simulink library "outp"  (R2021b)
(part 7 of 7)

  VNMM_NetworkReq_flg/1 -> VNMM_NetworkReq_flg_Inproc/1  "VNMM_NetworkReq_flg"
  VNMM_NetworkReq_flg_Inproc/1 -> UnitConverter226/1
  UnitConverter226/1 -> VOUTP_NetworkReq_flg/1  "VOUTP_NetworkReq_flg"
  VPMM_PowerUpState_enum/1 -> VPMM_PowerUpState_enum_Inproc/1  "VPMM_PowerUpState_enum"
  VPMM_PowerUpState_enum_Inproc/1 -> UnitConverter227/1
  UnitConverter227/1 -> VOUTP_PowerUpState_enum/1  "VOUTP_PowerUpState_enum"
  VPMM_PowerDownState_enum/1 -> VPMM_PowerDownState_enum_Inproc/1  "VPMM_PowerDownState_enum"
  VPMM_PowerDownState_enum_Inproc/1 -> UnitConverter228/1
  UnitConverter228/1 -> VOUTP_PowerDownState_enum/1  "VOUTP_PowerDownState_enum"
  VPMM_PowerUpFault_enum/1 -> VPMM_PowerUpFault_enum_Inproc/1  "VPMM_PowerUpFault_enum"
  VPMM_PowerUpFault_enum_Inproc/1 -> UnitConverter229/1
  UnitConverter229/1 -> VOUTP_PowerUpFault_enum/1  "VOUTP_PowerUpFault_enum"
  VPMM_PowerDownFault_enum/1 -> VPMM_PowerDownFault_enum_Inproc/1  "VPMM_PowerDownFault_enum"
  VPMM_PowerDownFault_enum_Inproc/1 -> UnitConverter230/1
  UnitConverter230/1 -> VOUTP_PowerDownFault_enum/1  "VOUTP_PowerDownFault_enum"
  VPMM_ActiveDischargeReq_flg/1 -> VPMM_ActiveDischargeReq_flg_Inproc/1  "VPMM_ActiveDischargeReq_flg"
  VPMM_ActiveDischargeReq_flg_Inproc/1 -> UnitConverter231/1
  UnitConverter231/1 -> VOUTP_ActiveDischargeReq_flg/1  "VOUTP_ActiveDischargeReq_flg"
  VPMM_DCDCEnaReq_flg/1 -> VPMM_DCDCEnaReq_flg_Inproc/1  "VPMM_DCDCEnaReq_flg"
  VPMM_DCDCEnaReq_flg_Inproc/1 -> UnitConverter232/1
  UnitConverter232/1 -> VOUTP_DCDCEnaReq_flg/1  "VOUTP_DCDCEnaReq_flg"
  VPMM_DCDCVoltSetpoint_V/1 -> VPMM_DCDCVoltSetpoint_V_Inproc/1  "VPMM_DCDCVoltSetpoint_V"
  VPMM_DCDCVoltSetpoint_V_Inproc/1 -> UnitConverter233/1
  UnitConverter233/1 -> VOUTP_DCDCVoltSetpoint_V/1  "VOUTP_DCDCVoltSetpoint_V"
  VPMM_HVBatCnctReq_flg/1 -> VPMM_HVBatCnctReq_flg_Inproc/1  "VPMM_HVBatCnctReq_flg"
  VPMM_HVBatCnctReq_flg_Inproc/1 -> UnitConverter234/1
  UnitConverter234/1 -> VOUTP_HVBatCnctReq_flg/1  "VOUTP_HVBatCnctReq_flg"
  VPMM_HVSysReadyToCharge_enum/1 -> VPMM_HVSysReadyToCharge_enum_Inproc/1  "VPMM_HVSysReadyToCharge_enum"
  VPMM_HVSysReadyToCharge_enum_Inproc/1 -> UnitConverter235/1
  UnitConverter235/1 -> VOUTP_HVSysReadyToCharge_enum/1  "VOUTP_HVSysReadyToCharge_enum"
  VPMM_PowerSta_enum/1 -> VPMM_PowerSta_enum_Inproc/1  "VPMM_PowerSta_enum"
  VPMM_PowerSta_enum_Inproc/1 -> UnitConverter236/1
  UnitConverter236/1 -> VOUTP_PowerSta_enum/1  "VOUTP_PowerSta_enum"
  VPMM_LVPwrSta_flg/1 -> VPMM_LVPwrSta_flg_Inproc/1  "VPMM_LVPwrSta_flg"
  VPMM_LVPwrSta_flg_Inproc/1 -> UnitConverter237/1
  UnitConverter237/1 -> VOUTP_LVPwrSta_flg/1  "VOUTP_LVPwrSta_flg"
  VPMM_HVPwrSta_flg/1 -> VPMM_HVPwrSta_flg_Inproc/1  "VPMM_HVPwrSta_flg"
  VPMM_HVPwrSta_flg_Inproc/1 -> UnitConverter238/1
  UnitConverter238/1 -> VOUTP_HVPwrSta_flg/1  "VOUTP_HVPwrSta_flg"
  VPMM_SysPowerMode_enum/1 -> VPMM_SysPowerMode_enum_Inproc/1  "VPMM_SysPowerMode_enum"
  VPMM_SysPowerMode_enum_Inproc/1 -> UnitConverter239/1
  UnitConverter239/1 -> VOUTP_SysPowerMode_enum/1  "VOUTP_SysPowerMode_enum"
  VPMM_FrMCUEnaReq_flg/1 -> VPMM_FrMCUEnaReq_flg_Inproc/1  "VPMM_FrMCUEnaReq_flg"
  VPMM_FrMCUEnaReq_flg_Inproc/1 -> UnitConverter240/1
  UnitConverter240/1 -> VOUTP_FrMCUEnaReq_flg/1  "VOUTP_FrMCUEnaReq_flg"
  VPMM_RrMCUEnaReq_flg/1 -> VPMM_RrMCUEnaReq_flg_Inproc/1  "VPMM_RrMCUEnaReq_flg"
  VPMM_RrMCUEnaReq_flg_Inproc/1 -> UnitConverter241/1
  UnitConverter241/1 -> VOUTP_RrMCUEnaReq_flg/1  "VOUTP_RrMCUEnaReq_flg"
  VPMM_DrivetrainSelect_enum/1 -> VPMM_DrivetrainSelect_enum_Inproc/1  "VPMM_DrivetrainSelect_enum"
  VPMM_DrivetrainSelect_enum_Inproc/1 -> UnitConverter242/1
  UnitConverter242/1 -> VOUTP_DrivetrainSelect_enum/1  "VOUTP_DrivetrainSelect_enum"
  VPMM_DrSeatSta_enum/1 -> VPMM_DrSeatSta_enum_Inproc/1  "VPMM_DrSeatSta_enum"
  VPMM_DrSeatSta_enum_Inproc/1 -> UnitConverter243/1
  UnitConverter243/1 -> VOUTP_DrSeatSta_enum/1  "VOUTP_DrSeatSta_enum"
  VPMM_PwrStaSelect_enum/1 -> VPMM_PwrStaSelect_enum_Inproc/1  "VPMM_PwrStaSelect_enum"
  VPMM_PwrStaSelect_enum_Inproc/1 -> UnitConverter244/1
  UnitConverter244/1 -> VOUTP_PwrStaSelect_enum/1  "VOUTP_PwrStaSelect_enum"
  VPMM_PwrStaConstraint_enum/1 -> VPMM_PwrStaConstraint_enum_Inproc/1  "VPMM_PwrStaConstraint_enum"
  VPMM_PwrStaConstraint_enum_Inproc/1 -> UnitConverter245/1
  UnitConverter245/1 -> VOUTP_PwrStaConstraint_enum/1  "VOUTP_PwrStaConstraint_enum"
  VPMM_TCountSta_enum/1 -> VPMM_TCountSta_enum_Inproc/1  "VPMM_TCountSta_enum"
  VPMM_TCountSta_enum_Inproc/1 -> UnitConverter246/1
  UnitConverter246/1 -> VOUTP_TCountSta_enum/1  "VOUTP_TCountSta_enum"
  VPMM_PwrUpReq_enum/1 -> VPMM_PwrUpReq_enum_Inproc/1  "VPMM_PwrUpReq_enum"
  VPMM_PwrUpReq_enum_Inproc/1 -> UnitConverter247/1
  UnitConverter247/1 -> VOUTP_PwrUpReq_enum/1  "VOUTP_PwrUpReq_enum"
  VPMM_PwrDownReq_enum/1 -> VPMM_PwrDownReq_enum_Inproc/1  "VPMM_PwrDownReq_enum"
  VPMM_PwrDownReq_enum_Inproc/1 -> UnitConverter248/1
  UnitConverter248/1 -> VOUTP_PwrDownReq_enum/1  "VOUTP_PwrDownReq_enum"
  VPMM_LowSOCWarn_enum/1 -> VPMM_LowSOCWarn_enum_Inproc/1  "VPMM_LowSOCWarn_enum"
  VPMM_LowSOCWarn_enum_Inproc/1 -> UnitConverter249/1
  UnitConverter249/1 -> VOUTP_LowSOCWarn_enum/1  "VOUTP_LowSOCWarn_enum"
  VPMM_ReVehThdChkSta_enum/1 -> VPMM_ReVehThdChkSta_enum_Inproc/1  "VPMM_ReVehThdChkSta_enum"
  VPMM_ReVehThdChkSta_enum_Inproc/1 -> UnitConverter250/1
  UnitConverter250/1 -> VOUTP_ReVehThdChkSta_enum/1  "VOUTP_ReVehThdChkSta_enum"
  VPMM_LVSysErrPwrOutErr_flg/1 -> VPMM_LVSysErrPwrOutErr_flg_Inproc/1  "VPMM_LVSysErrPwrOutErr_flg"
  VPMM_LVSysErrPwrOutErr_flg_Inproc/1 -> UnitConverter251/1
  UnitConverter251/1 -> VOUTP_LVSysErrPwrOutErr_flg/1  "VOUTP_LVSysErrPwrOutErr_flg"
  VPMM_EvccAplusPwrUpReq_flg/1 -> VPMM_EvccAplusPwrUpReq_flg_Inproc/1  "VPMM_EvccAplusPwrUpReq_flg"
  VPMM_EvccAplusPwrUpReq_flg_Inproc/1 -> UnitConverter252/1
  UnitConverter252/1 -> VOUTP_EvccAplusPwrUpReq_flg/1  "VOUTP_EvccAplusPwrUpReq_flg"
  VPMM_PwrStaONTOPopReq_flg/1 -> VPMM_PwrStaONTOPopReq_flg_Inproc/1  "VPMM_PwrStaONTOPopReq_flg"
  VPMM_PwrStaONTOPopReq_flg_Inproc/1 -> UnitConverter253/1
  UnitConverter253/1 -> VOUTP_PwrStaONTOPopReq_flg/1  "VOUTP_PwrStaONTOPopReq_flg"
  VPMM_IVIPwrStaONTOPopT_s/1 -> VPMM_IVIPwrStaONTOPopT_s_Inproc/1  "VPMM_IVIPwrStaONTOPopT_s"
  VPMM_IVIPwrStaONTOPopT_s_Inproc/1 -> UnitConverter254/1
  UnitConverter254/1 -> VOUTP_IVIPwrStaONTOPopT_s/1  "VOUTP_IVIPwrStaONTOPopT_s"
  VPMM_LVChrgHoldTtimer_s/1 -> VPMM_LVChrgHoldTtimer_s_Inproc/1  "VPMM_LVChrgHoldTtimer_s"
  VPMM_LVChrgHoldTtimer_s_Inproc/1 -> UnitConverter255/1
  UnitConverter255/1 -> VOUTP_LVChrgHoldTtimer_s/1  "VOUTP_LVChrgHoldTtimer_s"
  VPMM_LVBattChrgTimeCnt_s/1 -> VPMM_LVBattChrgTimeCnt_s_Inproc/1  "VPMM_LVBattChrgTimeCnt_s"
  VPMM_LVBattChrgTimeCnt_s_Inproc/1 -> UnitConverter256/1
  UnitConverter256/1 -> VOUTP_LVBattChrgTimeCnt_s/1  "VOUTP_LVBattChrgTimeCnt_s"
  VPMM_SilentChkAllowSleep_flg/1 -> VPMM_SilentChkAllowSleep_flg_Inproc/1  "VPMM_SilentChkAllowSleep_flg"
  VPMM_SilentChkAllowSleep_flg_Inproc/1 -> UnitConverter257/1
  UnitConverter257/1 -> VOUTP_SilentChkAllowSleep_flg/1  "VOUTP_SilentChkAllowSleep_flg"
  VPMM_TimerAllowSleep_flg/1 -> VPMM_TimerAllowSleep_flg_Inproc/1  "VPMM_TimerAllowSleep_flg"
  VPMM_TimerAllowSleep_flg_Inproc/1 -> UnitConverter258/1
  UnitConverter258/1 -> VOUTP_TimerAllowSleep_flg/1  "VOUTP_TimerAllowSleep_flg"
  VPMM_FDADC12VDetAvg_mV/1 -> VPMM_FDADC12VDetAvg_mV_Inproc/1  "VPMM_FDADC12VDetAvg_mV"
  VPMM_FDADC12VDetAvg_mV_Inproc/1 -> UnitConverter259/1
  UnitConverter259/1 -> VOUTP_FDADC12VDetAvg_mV/1  "VOUTP_FDADC12VDetAvg_mV"
  VPMM_PMMAllowECUSleep_flg/1 -> VPMM_PMMAllowECUSleep_flg_Inproc/1  "VPMM_PMMAllowECUSleep_flg"
  VPMM_PMMAllowECUSleep_flg_Inproc/1 -> UnitConverter260/1
  UnitConverter260/1 -> VOUTP_PMMAllowECUSleep_flg/1  "VOUTP_PMMAllowECUSleep_flg"
  VPMM_LVSilentChrgSta_enum/1 -> VPMM_LVSilentChrgSta_enum_Inproc/1  "VPMM_LVSilentChrgSta_enum"
  VPMM_LVSilentChrgSta_enum_Inproc/1 -> UnitConverter261/1
  UnitConverter261/1 -> VOUTP_LVSilentChrgSta_enum/1  "VOUTP_LVSilentChrgSta_enum"
  VPMM_LVSilentChrgReq_flg/1 -> VPMM_LVSilentChrgReq_flg_Inproc/1  "VPMM_LVSilentChrgReq_flg"
  VPMM_LVSilentChrgReq_flg_Inproc/1 -> UnitConverter262/1
  UnitConverter262/1 -> VOUTP_LVSilentChrgReq_flg/1  "VOUTP_LVSilentChrgReq_flg"
  VPMM_LVSilentChrgLv_enum/1 -> VPMM_LVSilentChrgLv_enum_Inproc/1  "VPMM_LVSilentChrgLv_enum"
  VPMM_LVSilentChrgLv_enum_Inproc/1 -> UnitConverter263/1
  UnitConverter263/1 -> VOUTP_LVSilentChrgLv_enum/1  "VOUTP_LVSilentChrgLv_enum"
  VPMM_CtrlFrPwrStbA1P_flg/1 -> VPMM_CtrlFrPwrStbA1P_flg_Inproc/1  "VPMM_CtrlFrPwrStbA1P_flg"
  VPMM_CtrlFrPwrStbA1P_flg_Inproc/1 -> UnitConverter264/1
  UnitConverter264/1 -> VOUTP_CtrlFrPwrStbA1P_flg/1  "VOUTP_CtrlFrPwrStbA1P_flg"
  VPMM_CtrlFrRC1_flg/1 -> VPMM_CtrlFrRC1_flg_Inproc/1  "VPMM_CtrlFrRC1_flg"
  VPMM_CtrlFrRC1_flg_Inproc/1 -> UnitConverter265/1
  UnitConverter265/1 -> VOUTP_CtrlFrRC1_flg/1  "VOUTP_CtrlFrRC1_flg"
  VPMM_CtrlFrBMSCCUCIR_flg/1 -> VPMM_CtrlFrBMSCCUCIR_flg_Inproc/1  "VPMM_CtrlFrBMSCCUCIR_flg"
  VPMM_CtrlFrBMSCCUCIR_flg_Inproc/1 -> UnitConverter266/1
  UnitConverter266/1 -> VOUTP_CtrlFrBMSCCUCIR_flg/1  "VOUTP_CtrlFrBMSCCUCIR_flg"
  VPMM_CtrlFrEDUINVERTER_flg/1 -> VPMM_CtrlFrEDUINVERTER_flg_Inproc/1  "VPMM_CtrlFrEDUINVERTER_flg"
  VPMM_CtrlFrEDUINVERTER_flg_Inproc/1 -> UnitConverter267/1
  UnitConverter267/1 -> VOUTP_CtrlFrEDUINVERTER_flg/1  "VOUTP_CtrlFrEDUINVERTER_flg"
  VPMM_HWResetSta_enum/1 -> VPMM_HWResetSta_enum_Inproc/1  "VPMM_HWResetSta_enum"
  VPMM_HWResetSta_enum_Inproc/1 -> UnitConverter268/1
  UnitConverter268/1 -> VOUTP_HWResetSta_enum/1  "VOUTP_HWResetSta_enum"
  VPMM_CtrlDrPwrStbA2_flg/1 -> VPMM_CtrlDrPwrStbA2_flg_Inproc/1  "VPMM_CtrlDrPwrStbA2_flg"
  VPMM_CtrlDrPwrStbA2_flg_Inproc/1 -> UnitConverter269/1
  UnitConverter269/1 -> VOUTP_CtrlDrPwrStbA2_flg/1  "VOUTP_CtrlDrPwrStbA2_flg"
  VPMM_PwrStaTOSta_enum/1 -> VPMM_PwrStaTOSta_enum_Inproc/1  "VPMM_PwrStaTOSta_enum"
  VPMM_PwrStaTOSta_enum_Inproc/1 -> UnitConverter270/1
  UnitConverter270/1 -> VOUTP_PwrStaTOSta_enum/1  "VOUTP_PwrStaTOSta_enum"
  VPMM_DCDCRlyDem_enum/1 -> VPMM_DCDCRlyDem_enum_Inproc/1  "VPMM_DCDCRlyDem_enum"
  VPMM_DCDCRlyDem_enum_Inproc/1 -> UnitConverter271/1
  UnitConverter271/1 -> VOUTP_DCDCRlyDem_enum/1  "VOUTP_DCDCRlyDem_enum"
  VPMM_EACRlyDem_enum/1 -> VPMM_EACRlyDem_enum_Inproc/1  "VPMM_EACRlyDem_enum"
  VPMM_EACRlyDem_enum_Inproc/1 -> UnitConverter272/1
  UnitConverter272/1 -> VOUTP_EACRlyDem_enum/1  "VOUTP_EACRlyDem_enum"
  VPMM_EHPSRlyDem_enum/1 -> VPMM_EHPSRlyDem_enum_Inproc/1  "VPMM_EHPSRlyDem_enum"
  VPMM_EHPSRlyDem_enum_Inproc/1 -> UnitConverter273/1
  UnitConverter273/1 -> VOUTP_EHPSRlyDem_enum/1  "VOUTP_EHPSRlyDem_enum"
  VPMM_DCDCEnDem_enum/1 -> VPMM_DCDCEnDem_enum_Inproc/1  "VPMM_DCDCEnDem_enum"
  VPMM_DCDCEnDem_enum_Inproc/1 -> UnitConverter274/1
  UnitConverter274/1 -> VOUTP_DCDCEnDem_enum/1  "VOUTP_DCDCEnDem_enum"
  VSCP_Vehspeed_kph/1 -> VSCP_Vehspeed_kph_Inproc/1  "VSCP_Vehspeed_kph"
  VSCP_Vehspeed_kph_Inproc/1 -> UnitConverter275/1
  UnitConverter275/1 -> VOUTP_Vehspeed_kph/1  "VOUTP_Vehspeed_kph"
  VSCP_SCPBrkSwSta_flg/1 -> VSCP_SCPBrkSwSta_flg_Inproc/1  "VSCP_SCPBrkSwSta_flg"
  VSCP_SCPBrkSwSta_flg_Inproc/1 -> UnitConverter276/1
  UnitConverter276/1 -> VOUTP_SCPBrkSwSta_flg/1  "VOUTP_SCPBrkSwSta_flg"
  VSCP_AmberWnlmpSta_flg/1 -> VSCP_AmberWnlmpSta_flg_Inproc/1  "VSCP_AmberWnlmpSta_flg"
  VSCP_AmberWnlmpSta_flg_Inproc/1 -> UnitConverter277/1
  UnitConverter277/1 -> VOUTP_AmberWnlmpSta_flg/1  "VOUTP_AmberWnlmpSta_flg"
  VSCP_ABSWnlmpSta_flg/1 -> VSCP_ABSWnlmpSta_flg_Inproc/1  "VSCP_ABSWnlmpSta_flg"
  VSCP_ABSWnlmpSta_flg_Inproc/1 -> UnitConverter278/1
  UnitConverter278/1 -> VOUTP_ABSWnlmpSta_flg/1  "VOUTP_ABSWnlmpSta_flg"
  VSCP_HSAFailed_flg/1 -> VSCP_HSAFailed_flg_Inproc/1  "VSCP_HSAFailed_flg"
  VSCP_HSAFailed_flg_Inproc/1 -> UnitConverter279/1
  UnitConverter279/1 -> VOUTP_HSAFailed_flg/1  "VOUTP_HSAFailed_flg"
  VSCP_MeterIndVehSpeed_kph/1 -> VSCP_MeterIndVehSpeed_kph_Inproc/1  "VSCP_MeterIndVehSpeed_kph"
  VSCP_MeterIndVehSpeed_kph_Inproc/1 -> UnitConverter280/1
  UnitConverter280/1 -> VOUTP_MeterIndVehSpeed_kph/1  "VOUTP_MeterIndVehSpeed_kph"
  VSCP_ABSFailed_flg/1 -> VSCP_ABSFailed_flg_Inproc/1  "VSCP_ABSFailed_flg"
  VSCP_ABSFailed_flg_Inproc/1 -> UnitConverter281/1
  UnitConverter281/1 -> VOUTP_ABSFailed_flg/1  "VOUTP_ABSFailed_flg"
  VSCP_ABSActive_flg/1 -> VSCP_ABSActive_flg_Inproc/1  "VSCP_ABSActive_flg"
  VSCP_ABSActive_flg_Inproc/1 -> UnitConverter282/1
  UnitConverter282/1 -> VOUTP_ABSActive_flg/1  "VOUTP_ABSActive_flg"
  VSCP_HSAActive_flg/1 -> VSCP_HSAActive_flg_Inproc/1  "VSCP_HSAActive_flg"
  VSCP_HSAActive_flg_Inproc/1 -> UnitConverter283/1
  UnitConverter283/1 -> VOUTP_HSAActive_flg/1  "VOUTP_HSAActive_flg"
  VSCP_RedWnlmpSta_flg/1 -> VSCP_RedWnlmpSta_flg_Inproc/1  "VSCP_RedWnlmpSta_flg"
  VSCP_RedWnlmpSta_flg_Inproc/1 -> UnitConverter284/1
  UnitConverter284/1 -> VOUTP_RedWnlmpSta_flg/1  "VOUTP_RedWnlmpSta_flg"
  VSCP_BrkPedalPos_pct/1 -> VSCP_BrkPedalPos_pct_Inproc/1  "VSCP_BrkPedalPos_pct"
  VSCP_BrkPedalPos_pct_Inproc/1 -> UnitConverter285/1
  UnitConverter285/1 -> VOUTP_BrkPedalPos_pct/1  "VOUTP_BrkPedalPos_pct"
  VSCP_OpenStatusOfDoor1_enum/1 -> VSCP_OpenStatusOfDoor1_enum_Inproc/1  "VSCP_OpenStatusOfDoor1_enum"
  VSCP_OpenStatusOfDoor1_enum_Inproc/1 -> UnitConverter286/1
  UnitConverter286/1 -> VOUTP_OpenStatusOfDoor1_enum/1  "VOUTP_OpenStatusOfDoor1_enum"
  VSCP_OpenStatusOfDoor2_enum/1 -> VSCP_OpenStatusOfDoor2_enum_Inproc/1  "VSCP_OpenStatusOfDoor2_enum"
  VSCP_OpenStatusOfDoor2_enum_Inproc/1 -> UnitConverter287/1
  UnitConverter287/1 -> VOUTP_OpenStatusOfDoor2_enum/1  "VOUTP_OpenStatusOfDoor2_enum"
  VSCP_SeatBeltSwitch_enum/1 -> VSCP_SeatBeltSwitch_enum_Inproc/1  "VSCP_SeatBeltSwitch_enum"
  VSCP_SeatBeltSwitch_enum_Inproc/1 -> UnitConverter288/1
  UnitConverter288/1 -> VOUTP_SeatBeltSwitch_enum/1  "VOUTP_SeatBeltSwitch_enum"
  VSCP_triggerBAM_flg/1 -> VSCP_triggerBAM_flg_Inproc/1  "VSCP_triggerBAM_flg"
  VSCP_triggerBAM_flg_Inproc/1 -> UnitConverter289/1
  UnitConverter289/1 -> VOUTP_triggerBAM_flg/1  "VOUTP_triggerBAM_flg"
  VSCP_CFGEM1Ctrl_raw/1 -> VSCP_CFGEM1Ctrl_raw_Inproc/1  "VSCP_CFGEM1Ctrl_raw"
  VSCP_CFGEM1Ctrl_raw_Inproc/1 -> UnitConverter290/1
  UnitConverter290/1 -> VOUTP_CFGEM1Ctrl_raw/1  "VOUTP_CFGEM1Ctrl_raw"
  VSCP_CFGEM1BAMTSize_raw/1 -> VSCP_CFGEM1BAMTSize_raw_Inproc/1  "VSCP_CFGEM1BAMTSize_raw"
  VSCP_CFGEM1BAMTSize_raw_Inproc/1 -> UnitConverter291/1
  UnitConverter291/1 -> VOUTP_CFGEM1BAMTSize_raw/1  "VOUTP_CFGEM1BAMTSize_raw"
  VSCP_CFGEM1BAMTNum_raw/1 -> VSCP_CFGEM1BAMTNum_raw_Inproc/1  "VSCP_CFGEM1BAMTNum_raw"
  VSCP_CFGEM1BAMTNum_raw_Inproc/1 -> UnitConverter292/1
  UnitConverter292/1 -> VOUTP_CFGEM1BAMTNum_raw/1  "VOUTP_CFGEM1BAMTNum_raw"
  VSCP_CFGEM1BAMRsv_raw/1 -> VSCP_CFGEM1BAMRsv_raw_Inproc/1  "VSCP_CFGEM1BAMRsv_raw"
  VSCP_CFGEM1BAMRsv_raw_Inproc/1 -> UnitConverter293/1
  UnitConverter293/1 -> VOUTP_CFGEM1BAMRsv_raw/1  "VOUTP_CFGEM1BAMRsv_raw"
  VSCP_CFGEM1BAMPGN_raw/1 -> VSCP_CFGEM1BAMPGN_raw_Inproc/1  "VSCP_CFGEM1BAMPGN_raw"
  VSCP_CFGEM1BAMPGN_raw_Inproc/1 -> UnitConverter294/1
  UnitConverter294/1 -> VOUTP_CFGEM1BAMPGN_raw/1  "VOUTP_CFGEM1BAMPGN_raw"
  VSCP_triggerDT_flg/1 -> VSCP_triggerDT_flg_Inproc/1  "VSCP_triggerDT_flg"
  VSCP_triggerDT_flg_Inproc/1 -> UnitConverter295/1
  UnitConverter295/1 -> VOUTP_triggerDT_flg/1  "VOUTP_triggerDT_flg"
  VSCP_DTbyte0_raw/1 -> VSCP_DTbyte0_raw_Inproc/1  "VSCP_DTbyte0_raw"
  VSCP_DTbyte0_raw_Inproc/1 -> UnitConverter296/1
  UnitConverter296/1 -> VOUTP_DTbyte0_raw/1  "VOUTP_DTbyte0_raw"
  VSCP_DTbyte1_raw/1 -> VSCP_DTbyte1_raw_Inproc/1  "VSCP_DTbyte1_raw"
  VSCP_DTbyte1_raw_Inproc/1 -> UnitConverter297/1
  UnitConverter297/1 -> VOUTP_DTbyte1_raw/1  "VOUTP_DTbyte1_raw"
  VSCP_DTbyte2_raw/1 -> VSCP_DTbyte2_raw_Inproc/1  "VSCP_DTbyte2_raw"
  VSCP_DTbyte2_raw_Inproc/1 -> UnitConverter298/1
  UnitConverter298/1 -> VOUTP_DTbyte2_raw/1  "VOUTP_DTbyte2_raw"
  VSCP_DTbyte3_raw/1 -> VSCP_DTbyte3_raw_Inproc/1  "VSCP_DTbyte3_raw"
  VSCP_DTbyte3_raw_Inproc/1 -> UnitConverter299/1
  UnitConverter299/1 -> VOUTP_DTbyte3_raw/1  "VOUTP_DTbyte3_raw"
  VSCP_DTbyte4_raw/1 -> VSCP_DTbyte4_raw_Inproc/1  "VSCP_DTbyte4_raw"
  VSCP_DTbyte4_raw_Inproc/1 -> UnitConverter300/1
  UnitConverter300/1 -> VOUTP_DTbyte4_raw/1  "VOUTP_DTbyte4_raw"
  VSCP_DTbyte5_raw/1 -> VSCP_DTbyte5_raw_Inproc/1  "VSCP_DTbyte5_raw"
  VSCP_DTbyte5_raw_Inproc/1 -> UnitConverter301/1
  UnitConverter301/1 -> VOUTP_DTbyte5_raw/1  "VOUTP_DTbyte5_raw"
  VSCP_DTbyte6_raw/1 -> VSCP_DTbyte6_raw_Inproc/1  "VSCP_DTbyte6_raw"
  VSCP_DTbyte6_raw_Inproc/1 -> UnitConverter302/1
  UnitConverter302/1 -> VOUTP_DTbyte6_raw/1  "VOUTP_DTbyte6_raw"
  VSCP_DTbyte7_raw/1 -> VSCP_DTbyte7_raw_Inproc/1  "VSCP_DTbyte7_raw"
  VSCP_DTbyte7_raw_Inproc/1 -> UnitConverter303/1
  UnitConverter303/1 -> VOUTP_DTbyte7_raw/1  "VOUTP_DTbyte7_raw"
  VSYS_HWVer1_cnt/1 -> VSYS_HWVer1_cnt_Inproc/1  "VSYS_HWVer1_cnt"
  VSYS_HWVer1_cnt_Inproc/1 -> UnitConverter304/1
  UnitConverter304/1 -> VOUTP_HWVer1_cnt/1  "VOUTP_HWVer1_cnt"
  VSYS_HWVer2_cnt/1 -> VSYS_HWVer2_cnt_Inproc/1  "VSYS_HWVer2_cnt"
  VSYS_HWVer2_cnt_Inproc/1 -> UnitConverter305/1
  UnitConverter305/1 -> VOUTP_HWVer2_cnt/1  "VOUTP_HWVer2_cnt"
  VSYS_HWVer3_cnt/1 -> VSYS_HWVer3_cnt_Inproc/1  "VSYS_HWVer3_cnt"
  VSYS_HWVer3_cnt_Inproc/1 -> UnitConverter306/1
  UnitConverter306/1 -> VOUTP_HWVer3_cnt/1  "VOUTP_HWVer3_cnt"
  VSYS_CarModel1_cnt/1 -> VSYS_CarModel1_cnt_Inproc/1  "VSYS_CarModel1_cnt"
  VSYS_CarModel1_cnt_Inproc/1 -> UnitConverter307/1
  UnitConverter307/1 -> VOUTP_CarModel1_cnt/1  "VOUTP_CarModel1_cnt"
  VSYS_CarModel2_cnt/1 -> VSYS_CarModel2_cnt_Inproc/1  "VSYS_CarModel2_cnt"
  VSYS_CarModel2_cnt_Inproc/1 -> UnitConverter308/1
  UnitConverter308/1 -> VOUTP_CarModel2_cnt/1  "VOUTP_CarModel2_cnt"
  VSYS_CarModel3_cnt/1 -> VSYS_CarModel3_cnt_Inproc/1  "VSYS_CarModel3_cnt"
  VSYS_CarModel3_cnt_Inproc/1 -> UnitConverter309/1
  UnitConverter309/1 -> VOUTP_CarModel3_cnt/1  "VOUTP_CarModel3_cnt"
  VSYS_ECU1_cnt/1 -> VSYS_ECU1_cnt_Inproc/1  "VSYS_ECU1_cnt"
  VSYS_ECU1_cnt_Inproc/1 -> UnitConverter310/1
  UnitConverter310/1 -> VOUTP_ECU1_cnt/1  "VOUTP_ECU1_cnt"
  VSYS_ECU2_cnt/1 -> VSYS_ECU2_cnt_Inproc/1  "VSYS_ECU2_cnt"
  VSYS_ECU2_cnt_Inproc/1 -> UnitConverter311/1
  UnitConverter311/1 -> VOUTP_ECU2_cnt/1  "VOUTP_ECU2_cnt"
  VSYS_Major1_cnt/1 -> VSYS_Major1_cnt_Inproc/1  "VSYS_Major1_cnt"
  VSYS_Major1_cnt_Inproc/1 -> UnitConverter312/1
  UnitConverter312/1 -> VOUTP_Major1_cnt/1  "VOUTP_Major1_cnt"
  VSYS_Major2_cnt/1 -> VSYS_Major2_cnt_Inproc/1  "VSYS_Major2_cnt"
  VSYS_Major2_cnt_Inproc/1 -> UnitConverter313/1
  UnitConverter313/1 -> VOUTP_Major2_cnt/1  "VOUTP_Major2_cnt"
  VSYS_Minor1_cnt/1 -> VSYS_Minor1_cnt_Inproc/1  "VSYS_Minor1_cnt"
  VSYS_Minor1_cnt_Inproc/1 -> UnitConverter314/1
  UnitConverter314/1 -> VOUTP_Minor1_cnt/1  "VOUTP_Minor1_cnt"
  VSYS_Minor2_cnt/1 -> VSYS_Minor2_cnt_Inproc/1  "VSYS_Minor2_cnt"
  VSYS_Minor2_cnt_Inproc/1 -> UnitConverter315/1
  UnitConverter315/1 -> VOUTP_Minor2_cnt/1  "VOUTP_Minor2_cnt"
  VSYS_Patch1_cnt/1 -> VSYS_Patch1_cnt_Inproc/1  "VSYS_Patch1_cnt"
  VSYS_Patch1_cnt_Inproc/1 -> UnitConverter316/1
  UnitConverter316/1 -> VOUTP_Patch1_cnt/1  "VOUTP_Patch1_cnt"
  VSYS_Patch2_cnt/1 -> VSYS_Patch2_cnt_Inproc/1  "VSYS_Patch2_cnt"
  VSYS_Patch2_cnt_Inproc/1 -> UnitConverter317/1
  UnitConverter317/1 -> VOUTP_Patch2_cnt/1  "VOUTP_Patch2_cnt"
  VSYS_Country1_cnt/1 -> VSYS_Country1_cnt_Inproc/1  "VSYS_Country1_cnt"
  VSYS_Country1_cnt_Inproc/1 -> UnitConverter318/1
  UnitConverter318/1 -> VOUTP_Country1_cnt/1  "VOUTP_Country1_cnt"
  VSYS_Country2_cnt/1 -> VSYS_Country2_cnt_Inproc/1  "VSYS_Country2_cnt"
  VSYS_Country2_cnt_Inproc/1 -> UnitConverter319/1
  UnitConverter319/1 -> VOUTP_Country2_cnt/1  "VOUTP_Country2_cnt"
  VSYS_Variation_cnt/1 -> VSYS_Variation_cnt_Inproc/1  "VSYS_Variation_cnt"
  VSYS_Variation_cnt_Inproc/1 -> UnitConverter320/1
  UnitConverter320/1 -> VOUTP_Variation_cnt/1  "VOUTP_Variation_cnt"
  VSYS_Dash1_cnt/1 -> VSYS_Dash1_cnt_Inproc/1  "VSYS_Dash1_cnt"
  VSYS_Dash1_cnt_Inproc/1 -> UnitConverter321/1
  UnitConverter321/1 -> VOUTP_Dash1_cnt/1  "VOUTP_Dash1_cnt"
  VSYS_Change1_cnt/1 -> VSYS_Change1_cnt_Inproc/1  "VSYS_Change1_cnt"
  VSYS_Change1_cnt_Inproc/1 -> UnitConverter322/1
  UnitConverter322/1 -> VOUTP_Change1_cnt/1  "VOUTP_Change1_cnt"
  VSYS_Change2_cnt/1 -> VSYS_Change2_cnt_Inproc/1  "VSYS_Change2_cnt"
  VSYS_Change2_cnt_Inproc/1 -> UnitConverter323/1
  UnitConverter323/1 -> VOUTP_Change2_cnt/1  "VOUTP_Change2_cnt"
  VSYS_Dash2_cnt/1 -> VSYS_Dash2_cnt_Inproc/1  "VSYS_Dash2_cnt"
  VSYS_Dash2_cnt_Inproc/1 -> UnitConverter324/1
  UnitConverter324/1 -> VOUTP_Dash2_cnt/1  "VOUTP_Dash2_cnt"
  VSYS_SHA1_cnt/1 -> VSYS_SHA1_cnt_Inproc/1  "VSYS_SHA1_cnt"
  VSYS_SHA1_cnt_Inproc/1 -> UnitConverter325/1
  UnitConverter325/1 -> VOUTP_SHA1_cnt/1  "VOUTP_SHA1_cnt"
  VSYS_SHA2_cnt/1 -> VSYS_SHA2_cnt_Inproc/1  "VSYS_SHA2_cnt"
  VSYS_SHA2_cnt_Inproc/1 -> UnitConverter326/1
  UnitConverter326/1 -> VOUTP_SHA2_cnt/1  "VOUTP_SHA2_cnt"
  VSYS_SHA3_cnt/1 -> VSYS_SHA3_cnt_Inproc/1  "VSYS_SHA3_cnt"
  VSYS_SHA3_cnt_Inproc/1 -> UnitConverter327/1
  UnitConverter327/1 -> VOUTP_SHA3_cnt/1  "VOUTP_SHA3_cnt"
  VSYS_SHA4_cnt/1 -> VSYS_SHA4_cnt_Inproc/1  "VSYS_SHA4_cnt"
  VSYS_SHA4_cnt_Inproc/1 -> UnitConverter328/1
  UnitConverter328/1 -> VOUTP_SHA4_cnt/1  "VOUTP_SHA4_cnt"
  VSYS_SHA5_cnt/1 -> VSYS_SHA5_cnt_Inproc/1  "VSYS_SHA5_cnt"
  VSYS_SHA5_cnt_Inproc/1 -> UnitConverter329/1
  UnitConverter329/1 -> VOUTP_SHA5_cnt/1  "VOUTP_SHA5_cnt"
  VSYS_SHA6_cnt/1 -> VSYS_SHA6_cnt_Inproc/1  "VSYS_SHA6_cnt"
  VSYS_SHA6_cnt_Inproc/1 -> UnitConverter330/1
  UnitConverter330/1 -> VOUTP_SHA6_cnt/1  "VOUTP_SHA6_cnt"
  VSYS_SHA7_cnt/1 -> VSYS_SHA7_cnt_Inproc/1  "VSYS_SHA7_cnt"
  VSYS_SHA7_cnt_Inproc/1 -> UnitConverter331/1
  UnitConverter331/1 -> VOUTP_SHA7_cnt/1  "VOUTP_SHA7_cnt"
  VSYS_SHA8_cnt/1 -> VSYS_SHA8_cnt_Inproc/1  "VSYS_SHA8_cnt"
  VSYS_SHA8_cnt_Inproc/1 -> UnitConverter332/1
  UnitConverter332/1 -> VOUTP_SHA8_cnt/1  "VOUTP_SHA8_cnt"
  VSYS_NvWriteReqRisingEdge_flg/1 -> VSYS_NvWriteReqRisingEdge_flg_Inproc/1  "VSYS_NvWriteReqRisingEdge_flg"
  VSYS_NvWriteReqRisingEdge_flg_Inproc/1 -> UnitConverter333/1
  UnitConverter333/1 -> VOUTP_NvWriteReqRisingEdge_flg/1  "VOUTP_NvWriteReqRisingEdge_flg"
  VSYS_FdcSlpReqRisingEdge_flg/1 -> VSYS_FdcSlpReqRisingEdge_flg_Inproc/1  "VSYS_FdcSlpReqRisingEdge_flg"
  VSYS_FdcSlpReqRisingEdge_flg_Inproc/1 -> UnitConverter334/1
  UnitConverter334/1 -> VOUTP_FdcSlpReqRisingEdge_flg/1  "VOUTP_FdcSlpReqRisingEdge_flg"
  VSYS_FdcSlpTime_sec/1 -> VSYS_FdcSlpTime_sec_Inproc/1  "VSYS_FdcSlpTime_sec"
  VSYS_FdcSlpTime_sec_Inproc/1 -> UnitConverter335/1
  UnitConverter335/1 -> VOUTP_FdcSlpTime_sec/1  "VOUTP_FdcSlpTime_sec"
  VSYS_PmicBootReason_enum/1 -> VSYS_PmicBootReason_enum_Inproc/1  "VSYS_PmicBootReason_enum"
  VSYS_PmicBootReason_enum_Inproc/1 -> UnitConverter336/1
  UnitConverter336/1 -> VOUTP_PmicBootReason_enum/1  "VOUTP_PmicBootReason_enum"
  VSYS_WisrBootReason_raw32/1 -> VSYS_WisrBootReason_raw32_Inproc/1  "VSYS_WisrBootReason_raw32"
  VSYS_WisrBootReason_raw32_Inproc/1 -> UnitConverter337/1
  UnitConverter337/1 -> VOUTP_WisrBootReason_raw32/1  "VOUTP_WisrBootReason_raw32"
  VSYS_AcoreRebootCmdACK_flg/1 -> VSYS_AcoreRebootCmdACK_flg_Inproc/1  "VSYS_AcoreRebootCmdACK_flg"
  VSYS_AcoreRebootCmdACK_flg_Inproc/1 -> UnitConverter338/1
  UnitConverter338/1 -> VOUTP_AcoreRebootCmdACK_flg/1  "VOUTP_AcoreRebootCmdACK_flg"
  VSYS_CurrentNmState_enum/1 -> VSYS_CurrentNmState_enum_Inproc/1  "VSYS_CurrentNmState_enum"
  VSYS_CurrentNmState_enum_Inproc/1 -> UnitConverter339/1
  UnitConverter339/1 -> VOUTP_CurrentNmState_enum/1  "VOUTP_CurrentNmState_enum"
  VTHC_FDCompCmd_rpm/1 -> VTHC_FDCompCmd_rpm_Inproc/1  "VTHC_FDCompCmd_rpm"
  VTHC_FDCompCmd_rpm_Inproc/1 -> UnitConverter340/1
  UnitConverter340/1 -> VOUTP_FDCompCmd_rpm/1  "VOUTP_FDCompCmd_rpm"
  VTHC_FDSOV1Cmd_flg/1 -> VTHC_FDSOV1Cmd_flg_Inproc/1  "VTHC_FDSOV1Cmd_flg"
  VTHC_FDSOV1Cmd_flg_Inproc/1 -> UnitConverter341/1
  UnitConverter341/1 -> VOUTP_FDSOV1Cmd_flg/1  "VOUTP_FDSOV1Cmd_flg"
  VTHC_FDSOV2Cmd_flg/1 -> VTHC_FDSOV2Cmd_flg_Inproc/1  "VTHC_FDSOV2Cmd_flg"
  VTHC_FDSOV2Cmd_flg_Inproc/1 -> UnitConverter342/1
  UnitConverter342/1 -> VOUTP_FDSOV2Cmd_flg/1  "VOUTP_FDSOV2Cmd_flg"
  VTHC_FDSOV3Cmd_flg/1 -> VTHC_FDSOV3Cmd_flg_Inproc/1  "VTHC_FDSOV3Cmd_flg"
  VTHC_FDSOV3Cmd_flg_Inproc/1 -> UnitConverter343/1
  UnitConverter343/1 -> VOUTP_FDSOV3Cmd_flg/1  "VOUTP_FDSOV3Cmd_flg"
  VTHC_FDEXV1Cmd_step/1 -> VTHC_FDEXV1Cmd_step_Inproc/1  "VTHC_FDEXV1Cmd_step"
  VTHC_FDEXV1Cmd_step_Inproc/1 -> UnitConverter344/1
  UnitConverter344/1 -> VOUTP_FDEXV1Cmd_step/1  "VOUTP_FDEXV1Cmd_step"
  VTHC_FDEXV2Cmd_step/1 -> VTHC_FDEXV2Cmd_step_Inproc/1  "VTHC_FDEXV2Cmd_step"
  VTHC_FDEXV2Cmd_step_Inproc/1 -> UnitConverter345/1
  UnitConverter345/1 -> VOUTP_FDEXV2Cmd_step/1  "VOUTP_FDEXV2Cmd_step"
  VTHC_FDSOTXVCmd_flg/1 -> VTHC_FDSOTXVCmd_flg_Inproc/1  "VTHC_FDSOTXVCmd_flg"
  VTHC_FDSOTXVCmd_flg_Inproc/1 -> UnitConverter346/1
  UnitConverter346/1 -> VOUTP_FDSOTXVCmd_flg/1  "VOUTP_FDSOTXVCmd_flg"
  VTHC_FDFWVCmd_flg/1 -> VTHC_FDFWVCmd_flg_Inproc/1  "VTHC_FDFWVCmd_flg"
  VTHC_FDFWVCmd_flg_Inproc/1 -> UnitConverter347/1
  UnitConverter347/1 -> VOUTP_FDFWVCmd_flg/1  "VOUTP_FDFWVCmd_flg"
  VTHC_FDTWVCmd_pct/1 -> VTHC_FDTWVCmd_pct_Inproc/1  "VTHC_FDTWVCmd_pct"
  VTHC_FDTWVCmd_pct_Inproc/1 -> UnitConverter348/1
  UnitConverter348/1 -> VOUTP_FDTWVCmd_pct/1  "VOUTP_FDTWVCmd_pct"
  VTHC_FDFrWPTCHeatPwrCmd_W/1 -> VTHC_FDFrWPTCHeatPwrCmd_W_Inproc/1  "VTHC_FDFrWPTCHeatPwrCmd_W"
  VTHC_FDFrWPTCHeatPwrCmd_W_Inproc/1 -> UnitConverter349/1
  UnitConverter349/1 -> VOUTP_FDFrWPTCHeatPwrCmd_W/1  "VOUTP_FDFrWPTCHeatPwrCmd_W"
  VTHC_CoolgFanActDuty_pct/1 -> VTHC_CoolgFanActDuty_pct_Inproc/1  "VTHC_CoolgFanActDuty_pct"
  VTHC_CoolgFanActDuty_pct_Inproc/1 -> UnitConverter350/1
  UnitConverter350/1 -> VOUTP_CoolgFanActDuty_pct/1  "VOUTP_CoolgFanActDuty_pct"
  VTHC_FDAGSCmd_enum/1 -> VTHC_FDAGSCmd_enum_Inproc/1  "VTHC_FDAGSCmd_enum"
  VTHC_FDAGSCmd_enum_Inproc/1 -> UnitConverter351/1
  UnitConverter351/1 -> VOUTP_FDAGSCmd_enum/1  "VOUTP_FDAGSCmd_enum"
  VTHC_FDEWP1Cmd_enum/1 -> VTHC_FDEWP1Cmd_enum_Inproc/1  "VTHC_FDEWP1Cmd_enum"
  VTHC_FDEWP1Cmd_enum_Inproc/1 -> UnitConverter352/1
  UnitConverter352/1 -> VOUTP_FDEWP1Cmd_enum/1  "VOUTP_FDEWP1Cmd_enum"
  VTHC_FDEWP2Cmd_enum/1 -> VTHC_FDEWP2Cmd_enum_Inproc/1  "VTHC_FDEWP2Cmd_enum"
  VTHC_FDEWP2Cmd_enum_Inproc/1 -> UnitConverter353/1
  UnitConverter353/1 -> VOUTP_FDEWP2Cmd_enum/1  "VOUTP_FDEWP2Cmd_enum"
  VTHC_FDEWP3Cmd_enum/1 -> VTHC_FDEWP3Cmd_enum_Inproc/1  "VTHC_FDEWP3Cmd_enum"
  VTHC_FDEWP3Cmd_enum_Inproc/1 -> UnitConverter354/1
  UnitConverter354/1 -> VOUTP_FDEWP3Cmd_enum/1  "VOUTP_FDEWP3Cmd_enum"
  VTHC_FDFrLeAPTCHeatPwrCmd_W/1 -> VTHC_FDFrLeAPTCHeatPwrCmd_W_Inproc/1  "VTHC_FDFrLeAPTCHeatPwrCmd_W"
  VTHC_FDFrLeAPTCHeatPwrCmd_W_Inproc/1 -> UnitConverter355/1
  UnitConverter355/1 -> VOUTP_FDFrLeAPTCHeatPwrCmd_W/1  "VOUTP_FDFrLeAPTCHeatPwrCmd_W"
  VTHC_FDFrRiAPTCHeatPwrCmd_W/1 -> VTHC_FDFrRiAPTCHeatPwrCmd_W_Inproc/1  "VTHC_FDFrRiAPTCHeatPwrCmd_W"
  VTHC_FDFrRiAPTCHeatPwrCmd_W_Inproc/1 -> UnitConverter356/1
  UnitConverter356/1 -> VOUTP_FDFrRiAPTCHeatPwrCmd_W/1  "VOUTP_FDFrRiAPTCHeatPwrCmd_W"
  VTHC_FDRrAPTCHeatPwrCmd_W/1 -> VTHC_FDRrAPTCHeatPwrCmd_W_Inproc/1  "VTHC_FDRrAPTCHeatPwrCmd_W"
  VTHC_FDRrAPTCHeatPwrCmd_W_Inproc/1 -> UnitConverter357/1
  UnitConverter357/1 -> VOUTP_FDRrAPTCHeatPwrCmd_W/1  "VOUTP_FDRrAPTCHeatPwrCmd_W"
  VTHC_FDBlowerCmd_pct/1 -> VTHC_FDBlowerCmd_pct_Inproc/1  "VTHC_FDBlowerCmd_pct"
  VTHC_FDBlowerCmd_pct_Inproc/1 -> UnitConverter358/1
  UnitConverter358/1 -> VOUTP_FDBlowerCmd_pct/1  "VOUTP_FDBlowerCmd_pct"
  VTHC_BatteryMode_enum/1 -> VTHC_BatteryMode_enum_Inproc/1  "VTHC_BatteryMode_enum"
  VTHC_BatteryMode_enum_Inproc/1 -> UnitConverter359/1
  UnitConverter359/1 -> VOUTP_BatteryMode_enum/1  "VOUTP_BatteryMode_enum"
  VTHC_EDriveMode_enum/1 -> VTHC_EDriveMode_enum_Inproc/1  "VTHC_EDriveMode_enum"
  VTHC_EDriveMode_enum_Inproc/1 -> UnitConverter360/1
  UnitConverter360/1 -> VOUTP_EDriveMode_enum/1  "VOUTP_EDriveMode_enum"
  VTHC_CabinMode_enum/1 -> VTHC_CabinMode_enum_Inproc/1  "VTHC_CabinMode_enum"
  VTHC_CabinMode_enum_Inproc/1 -> UnitConverter361/1
  UnitConverter361/1 -> VOUTP_CabinMode_enum/1  "VOUTP_CabinMode_enum"
  VTHC_CCUACLampSts_flg/1 -> VTHC_CCUACLampSts_flg_Inproc/1  "VTHC_CCUACLampSts_flg"
  VTHC_CCUACLampSts_flg_Inproc/1 -> UnitConverter362/1
  UnitConverter362/1 -> VOUTP_CCUACLampSts_flg/1  "VOUTP_CCUACLampSts_flg"
  VTHC_CCUAutoLampSts_flg/1 -> VTHC_CCUAutoLampSts_flg_Inproc/1  "VTHC_CCUAutoLampSts_flg"
  VTHC_CCUAutoLampSts_flg_Inproc/1 -> UnitConverter363/1
  UnitConverter363/1 -> VOUTP_CCUAutoLampSts_flg/1  "VOUTP_CCUAutoLampSts_flg"
  VTHC_CCUACMaxLampSts_flg/1 -> VTHC_CCUACMaxLampSts_flg_Inproc/1  "VTHC_CCUACMaxLampSts_flg"
  VTHC_CCUACMaxLampSts_flg_Inproc/1 -> UnitConverter364/1
  UnitConverter364/1 -> VOUTP_CCUACMaxLampSts_flg/1  "VOUTP_CCUACMaxLampSts_flg"
  VTHC_CCUSyncLampSts_flg/1 -> VTHC_CCUSyncLampSts_flg_Inproc/1  "VTHC_CCUSyncLampSts_flg"
  VTHC_CCUSyncLampSts_flg_Inproc/1 -> UnitConverter365/1
  UnitConverter365/1 -> VOUTP_CCUSyncLampSts_flg/1  "VOUTP_CCUSyncLampSts_flg"
  VTHC_sigAirIntenZon1St_enum/1 -> VTHC_sigAirIntenZon1St_enum_Inproc/1  "VTHC_sigAirIntenZon1St_enum"
  VTHC_sigAirIntenZon1St_enum_Inproc/1 -> UnitConverter366/1
  UnitConverter366/1 -> VOUTP_sigAirIntenZon1St_enum/1  "VOUTP_sigAirIntenZon1St_enum"
  VTHC_sigWindDirZon1St_enum/1 -> VTHC_sigWindDirZon1St_enum_Inproc/1  "VTHC_sigWindDirZon1St_enum"
  VTHC_sigWindDirZon1St_enum_Inproc/1 -> UnitConverter367/1
  UnitConverter367/1 -> VOUTP_sigWindDirZon1St_enum/1  "VOUTP_sigWindDirZon1St_enum"
  VTHC_sigRecircSt_flg/1 -> VTHC_sigRecircSt_flg_Inproc/1  "VTHC_sigRecircSt_flg"
  VTHC_sigRecircSt_flg_Inproc/1 -> UnitConverter368/1
  UnitConverter368/1 -> VOUTP_sigRecircSt_flg/1  "VOUTP_sigRecircSt_flg"
  VTHC_sigSetTempZon1St_C/1 -> VTHC_sigSetTempZon1St_C_Inproc/1  "VTHC_sigSetTempZon1St_C"
  VTHC_sigSetTempZon1St_C_Inproc/1 -> UnitConverter369/1
  UnitConverter369/1 -> VOUTP_sigSetTempZon1St_C/1  "VOUTP_sigSetTempZon1St_C"
  VTHC_sigSetTempZon2St_C/1 -> VTHC_sigSetTempZon2St_C_Inproc/1  "VTHC_sigSetTempZon2St_C"
  VTHC_sigSetTempZon2St_C_Inproc/1 -> UnitConverter370/1
  UnitConverter370/1 -> VOUTP_sigSetTempZon2St_C/1  "VOUTP_sigSetTempZon2St_C"
  VTHC_sigClntTHvBattOut_C/1 -> VTHC_sigClntTHvBattOut_C_Inproc/1  "VTHC_sigClntTHvBattOut_C"
  VTHC_sigClntTHvBattOut_C_Inproc/1 -> UnitConverter371/1
  UnitConverter371/1 -> VOUTP_sigClntTHvBattOut_C/1  "VOUTP_sigClntTHvBattOut_C"
  VTHC_sigCbnSolarLeft_W/1 -> VTHC_sigCbnSolarLeft_W_Inproc/1  "VTHC_sigCbnSolarLeft_W"
  VTHC_sigCbnSolarLeft_W_Inproc/1 -> UnitConverter372/1
  UnitConverter372/1 -> VOUTP_sigCbnSolarLeft_W/1  "VOUTP_sigCbnSolarLeft_W"
  VTHC_sigClntTHvBattIn_C/1 -> VTHC_sigClntTHvBattIn_C_Inproc/1  "VTHC_sigClntTHvBattIn_C"
  VTHC_sigClntTHvBattIn_C_Inproc/1 -> UnitConverter373/1
  UnitConverter373/1 -> VOUTP_sigClntTHvBattIn_C/1  "VOUTP_sigClntTHvBattIn_C"
  VTHC_sigCbnSolarRight_W/1 -> VTHC_sigCbnSolarRight_W_Inproc/1  "VTHC_sigCbnSolarRight_W"
  VTHC_sigCbnSolarRight_W_Inproc/1 -> UnitConverter374/1
  UnitConverter374/1 -> VOUTP_sigCbnSolarRight_W/1  "VOUTP_sigCbnSolarRight_W"
  VTHC_sigAmbAirT_C/1 -> VTHC_sigAmbAirT_C_Inproc/1  "VTHC_sigAmbAirT_C"
  VTHC_sigAmbAirT_C_Inproc/1 -> UnitConverter375/1
  UnitConverter375/1 -> VOUTP_sigAmbAirT_C/1  "VOUTP_sigAmbAirT_C"
  VTHC_sigCbnAirT_C/1 -> VTHC_sigCbnAirT_C_Inproc/1  "VTHC_sigCbnAirT_C"
  VTHC_sigCbnAirT_C_Inproc/1 -> UnitConverter376/1
  UnitConverter376/1 -> VOUTP_sigCbnAirT_C/1  "VOUTP_sigCbnAirT_C"
  VTHC_ACSubMode_enum/1 -> VTHC_ACSubMode_enum_Inproc/1  "VTHC_ACSubMode_enum"
  VTHC_ACSubMode_enum_Inproc/1 -> UnitConverter377/1
  UnitConverter377/1 -> VOUTP_ACSubMode_enum/1  "VOUTP_ACSubMode_enum"
  VTHC_FDRecyAutoCmd_enum/1 -> VTHC_FDRecyAutoCmd_enum_Inproc/1  "VTHC_FDRecyAutoCmd_enum"
  VTHC_FDRecyAutoCmd_enum_Inproc/1 -> UnitConverter378/1
  UnitConverter378/1 -> VOUTP_FDRecyAutoCmd_enum/1  "VOUTP_FDRecyAutoCmd_enum"
  VTHC_ACModeMem_enum/1 -> VTHC_ACModeMem_enum_Inproc/1  "VTHC_ACModeMem_enum"
  VTHC_ACModeMem_enum_Inproc/1 -> UnitConverter379/1
  UnitConverter379/1 -> VOUTP_ACModeMem_enum/1  "VOUTP_ACModeMem_enum"
  VTHC_Face_flg/1 -> VTHC_Face_flg_Inproc/1  "VTHC_Face_flg"
  VTHC_Face_flg_Inproc/1 -> UnitConverter380/1
  UnitConverter380/1 -> VOUTP_Face_flg/1  "VOUTP_Face_flg"
  VTHC_Foot_flg/1 -> VTHC_Foot_flg_Inproc/1  "VTHC_Foot_flg"
  VTHC_Foot_flg_Inproc/1 -> UnitConverter381/1
  UnitConverter381/1 -> VOUTP_Foot_flg/1  "VOUTP_Foot_flg"
  VTHC_Frost_flg/1 -> VTHC_Frost_flg_Inproc/1  "VTHC_Frost_flg"
  VTHC_Frost_flg_Inproc/1 -> UnitConverter382/1
  UnitConverter382/1 -> VOUTP_Frost_flg/1  "VOUTP_Frost_flg"
  VTHC_FaceM_flg/1 -> VTHC_FaceM_flg_Inproc/1  "VTHC_FaceM_flg"
  VTHC_FaceM_flg_Inproc/1 -> UnitConverter383/1
  UnitConverter383/1 -> VOUTP_FaceM_flg/1  "VOUTP_FaceM_flg"
  VTHC_FootM_flg/1 -> VTHC_FootM_flg_Inproc/1  "VTHC_FootM_flg"
  VTHC_FootM_flg_Inproc/1 -> UnitConverter384/1
  UnitConverter384/1 -> VOUTP_FootM_flg/1  "VOUTP_FootM_flg"
  VTHC_CCUSyncSts_flg/1 -> VTHC_CCUSyncSts_flg_Inproc/1  "VTHC_CCUSyncSts_flg"
  VTHC_CCUSyncSts_flg_Inproc/1 -> UnitConverter385/1
  UnitConverter385/1 -> VOUTP_CCUSyncSts_flg/1  "VOUTP_CCUSyncSts_flg"
  VTHC_ACForceOFF_flg/1 -> VTHC_ACForceOFF_flg_Inproc/1  "VTHC_ACForceOFF_flg"
  VTHC_ACForceOFF_flg_Inproc/1 -> UnitConverter386/1
  UnitConverter386/1 -> VOUTP_ACForceOFF_flg/1  "VOUTP_ACForceOFF_flg"
  VTHC_RecAutoFlg_flg/1 -> VTHC_RecAutoFlg_flg_Inproc/1  "VTHC_RecAutoFlg_flg"
  VTHC_RecAutoFlg_flg_Inproc/1 -> UnitConverter387/1
  UnitConverter387/1 -> VOUTP_RecAutoFlg_flg/1  "VOUTP_RecAutoFlg_flg"
  VTHC_AirIntenZone1M_enum/1 -> VTHC_AirIntenZone1M_enum_Inproc/1  "VTHC_AirIntenZone1M_enum"
  VTHC_AirIntenZone1M_enum_Inproc/1 -> UnitConverter388/1
  UnitConverter388/1 -> VOUTP_AirIntenZone1M_enum/1  "VOUTP_AirIntenZone1M_enum"
  VTHC_fdefog_flg/1 -> VTHC_fdefog_flg_Inproc/1  "VTHC_fdefog_flg"
  VTHC_fdefog_flg_Inproc/1 -> UnitConverter389/1
  UnitConverter389/1 -> VOUTP_fdefog_flg/1  "VOUTP_fdefog_flg"
  VTHC_sigSetTempZon2StM_C/1 -> VTHC_sigSetTempZon2StM_C_Inproc/1  "VTHC_sigSetTempZon2StM_C"
  VTHC_sigSetTempZon2StM_C_Inproc/1 -> UnitConverter390/1
  UnitConverter390/1 -> VOUTP_sigSetTempZon2StM_C/1  "VOUTP_sigSetTempZon2StM_C"
  VTHC_FDCTHCMAPTCWarningSta_flg/1 -> VTHC_FDCTHCMAPTCWarningSta_flg_Inproc/1  "VTHC_FDCTHCMAPTCWarningSta_flg"
  VTHC_FDCTHCMAPTCWarningSta_flg_Inproc/1 -> UnitConverter391/1
  UnitConverter391/1 -> VOUTP_FDCTHCMAPTCWarningSta_flg/1  "VOUTP_FDCTHCMAPTCWarningSta_flg"
  VTPM_LFBatWarn_flg/1 -> VTPM_LFBatWarn_flg_Inproc/1  "VTPM_LFBatWarn_flg"
  VTPM_LFBatWarn_flg_Inproc/1 -> UnitConverter392/1
  UnitConverter392/1 -> VOUTP_LFBatWarn_flg/1  "VOUTP_LFBatWarn_flg"
  VTPM_RFBatWarn_flg/1 -> VTPM_RFBatWarn_flg_Inproc/1  "VTPM_RFBatWarn_flg"
  VTPM_RFBatWarn_flg_Inproc/1 -> UnitConverter393/1
  UnitConverter393/1 -> VOUTP_RFBatWarn_flg/1  "VOUTP_RFBatWarn_flg"
  VTPM_LRBatWarn_flg/1 -> VTPM_LRBatWarn_flg_Inproc/1  "VTPM_LRBatWarn_flg"
  VTPM_LRBatWarn_flg_Inproc/1 -> UnitConverter394/1
  UnitConverter394/1 -> VOUTP_LRBatWarn_flg/1  "VOUTP_LRBatWarn_flg"
  VTPM_RRBatWarn_flg/1 -> VTPM_RRBatWarn_flg_Inproc/1  "VTPM_RRBatWarn_flg"
  VTPM_RRBatWarn_flg_Inproc/1 -> UnitConverter395/1
  UnitConverter395/1 -> VOUTP_RRBatWarn_flg/1  "VOUTP_RRBatWarn_flg"
  VTPM_LFWheelPress_raw8/1 -> VTPM_LFWheelPress_raw8_Inproc/1  "VTPM_LFWheelPress_raw8"
  VTPM_LFWheelPress_raw8_Inproc/1 -> UnitConverter396/1
  UnitConverter396/1 -> VOUTP_LFWheelPress_raw8/1  "VOUTP_LFWheelPress_raw8"
  VTPM_RFWheelPress_raw8/1 -> VTPM_RFWheelPress_raw8_Inproc/1  "VTPM_RFWheelPress_raw8"
  VTPM_RFWheelPress_raw8_Inproc/1 -> UnitConverter397/1
  UnitConverter397/1 -> VOUTP_RFWheelPress_raw8/1  "VOUTP_RFWheelPress_raw8"
  VTPM_LRWheelPress_raw8/1 -> VTPM_LRWheelPress_raw8_Inproc/1  "VTPM_LRWheelPress_raw8"
  VTPM_LRWheelPress_raw8_Inproc/1 -> UnitConverter398/1
  UnitConverter398/1 -> VOUTP_LRWheelPress_raw8/1  "VOUTP_LRWheelPress_raw8"
  VTPM_RRWheelPress_raw8/1 -> VTPM_RRWheelPress_raw8_Inproc/1  "VTPM_RRWheelPress_raw8"
  VTPM_RRWheelPress_raw8_Inproc/1 -> UnitConverter399/1
  UnitConverter399/1 -> VOUTP_RRWheelPress_raw8/1  "VOUTP_RRWheelPress_raw8"
  VTPM_LFWheelTemp_C/1 -> VTPM_LFWheelTemp_C_Inproc/1  "VTPM_LFWheelTemp_C"
  VTPM_LFWheelTemp_C_Inproc/1 -> UnitConverter400/1
  UnitConverter400/1 -> VOUTP_LFWheelTemp_C/1  "VOUTP_LFWheelTemp_C"
  VTPM_RFWheelTemp_C/1 -> VTPM_RFWheelTemp_C_Inproc/1  "VTPM_RFWheelTemp_C"
  VTPM_RFWheelTemp_C_Inproc/1 -> UnitConverter401/1
  UnitConverter401/1 -> VOUTP_RFWheelTemp_C/1  "VOUTP_RFWheelTemp_C"
  VTPM_LRWheelTemp_C/1 -> VTPM_LRWheelTemp_C_Inproc/1  "VTPM_LRWheelTemp_C"
  VTPM_LRWheelTemp_C_Inproc/1 -> UnitConverter402/1
  UnitConverter402/1 -> VOUTP_LRWheelTemp_C/1  "VOUTP_LRWheelTemp_C"
  VTPM_RRWheelTemp_C/1 -> VTPM_RRWheelTemp_C_Inproc/1  "VTPM_RRWheelTemp_C"
  VTPM_RRWheelTemp_C_Inproc/1 -> UnitConverter403/1
  UnitConverter403/1 -> VOUTP_RRWheelTemp_C/1  "VOUTP_RRWheelTemp_C"
  VTPM_LFSensorFail_flg/1 -> VTPM_LFSensorFail_flg_Inproc/1  "VTPM_LFSensorFail_flg"
  VTPM_LFSensorFail_flg_Inproc/1 -> UnitConverter404/1
  UnitConverter404/1 -> VOUTP_LFSensorFail_flg/1  "VOUTP_LFSensorFail_flg"
  VTPM_RFSensorFail_flg/1 -> VTPM_RFSensorFail_flg_Inproc/1  "VTPM_RFSensorFail_flg"
  VTPM_RFSensorFail_flg_Inproc/1 -> UnitConverter405/1
  UnitConverter405/1 -> VOUTP_RFSensorFail_flg/1  "VOUTP_RFSensorFail_flg"
  VTPM_LRSensorFail_flg/1 -> VTPM_LRSensorFail_flg_Inproc/1  "VTPM_LRSensorFail_flg"
  VTPM_LRSensorFail_flg_Inproc/1 -> UnitConverter406/1
  UnitConverter406/1 -> VOUTP_LRSensorFail_flg/1  "VOUTP_LRSensorFail_flg"
  VTPM_RRSensorFail_flg/1 -> VTPM_RRSensorFail_flg_Inproc/1  "VTPM_RRSensorFail_flg"
  VTPM_RRSensorFail_flg_Inproc/1 -> UnitConverter407/1
  UnitConverter407/1 -> VOUTP_RRSensorFail_flg/1  "VOUTP_RRSensorFail_flg"
  VTPM_LFWheelDebug_flg/1 -> VTPM_LFWheelDebug_flg_Inproc/1  "VTPM_LFWheelDebug_flg"
  VTPM_LFWheelDebug_flg_Inproc/1 -> UnitConverter408/1
  UnitConverter408/1 -> VOUTP_LFWheelDebug_flg/1  "VOUTP_LFWheelDebug_flg"
  VTPM_LRWheelDebug_flg/1 -> VTPM_LRWheelDebug_flg_Inproc/1  "VTPM_LRWheelDebug_flg"
  VTPM_LRWheelDebug_flg_Inproc/1 -> UnitConverter409/1
  UnitConverter409/1 -> VOUTP_LRWheelDebug_flg/1  "VOUTP_LRWheelDebug_flg"
  VTPM_RFWheelDebug_flg/1 -> VTPM_RFWheelDebug_flg_Inproc/1  "VTPM_RFWheelDebug_flg"
  VTPM_RFWheelDebug_flg_Inproc/1 -> UnitConverter410/1
  UnitConverter410/1 -> VOUTP_RFWheelDebug_flg/1  "VOUTP_RFWheelDebug_flg"
  VTPM_RRWheelDebug_flg/1 -> VTPM_RRWheelDebug_flg_Inproc/1  "VTPM_RRWheelDebug_flg"
  VTPM_RRWheelDebug_flg_Inproc/1 -> UnitConverter411/1
  UnitConverter411/1 -> VOUTP_RRWheelDebug_flg/1  "VOUTP_RRWheelDebug_flg"
  VTPM_TPMSResButtAllow_flg/1 -> VTPM_TPMSResButtAllow_flg_Inproc/1  "VTPM_TPMSResButtAllow_flg"
  VTPM_TPMSResButtAllow_flg_Inproc/1 -> UnitConverter412/1
  UnitConverter412/1 -> VOUTP_TPMSResButtAllow_flg/1  "VOUTP_TPMSResButtAllow_flg"
  VTPM_TPMSCaliButtAllow_flg/1 -> VTPM_TPMSCaliButtAllow_flg_Inproc/1  "VTPM_TPMSCaliButtAllow_flg"
  VTPM_TPMSCaliButtAllow_flg_Inproc/1 -> UnitConverter413/1
  UnitConverter413/1 -> VOUTP_TPMSCaliButtAllow_flg/1  "VOUTP_TPMSCaliButtAllow_flg"
  VTPM_LFPressIndi_enum/1 -> VTPM_LFPressIndi_enum_Inproc/1  "VTPM_LFPressIndi_enum"
  VTPM_LFPressIndi_enum_Inproc/1 -> UnitConverter414/1
  UnitConverter414/1 -> VOUTP_LFPressIndi_enum/1  "VOUTP_LFPressIndi_enum"
  VTPM_RFPressIndi_enum/1 -> VTPM_RFPressIndi_enum_Inproc/1  "VTPM_RFPressIndi_enum"
  VTPM_RFPressIndi_enum_Inproc/1 -> UnitConverter415/1
  UnitConverter415/1 -> VOUTP_RFPressIndi_enum/1  "VOUTP_RFPressIndi_enum"
  VTPM_LRPressIndi_enum/1 -> VTPM_LRPressIndi_enum_Inproc/1  "VTPM_LRPressIndi_enum"
  VTPM_LRPressIndi_enum_Inproc/1 -> UnitConverter416/1
  UnitConverter416/1 -> VOUTP_LRPressIndi_enum/1  "VOUTP_LRPressIndi_enum"
  VTPM_RRPressIndi_enum/1 -> VTPM_RRPressIndi_enum_Inproc/1  "VTPM_RRPressIndi_enum"
  VTPM_RRPressIndi_enum_Inproc/1 -> UnitConverter417/1
  UnitConverter417/1 -> VOUTP_RRPressIndi_enum/1  "VOUTP_RRPressIndi_enum"
  VTPM_TPMSWarnIndi_enum/1 -> VTPM_TPMSWarnIndi_enum_Inproc/1  "VTPM_TPMSWarnIndi_enum"
  VTPM_TPMSWarnIndi_enum_Inproc/1 -> UnitConverter418/1
  UnitConverter418/1 -> VOUTP_TPMSWarnIndi_enum/1  "VOUTP_TPMSWarnIndi_enum"
  VTPM_LFWheelTmpIndi_flg/1 -> VTPM_LFWheelTmpIndi_flg_Inproc/1  "VTPM_LFWheelTmpIndi_flg"
  VTPM_LFWheelTmpIndi_flg_Inproc/1 -> UnitConverter419/1
  UnitConverter419/1 -> VOUTP_LFWheelTmpIndi_flg/1  "VOUTP_LFWheelTmpIndi_flg"
  VTPM_RFWheelTmpIndi_flg/1 -> VTPM_RFWheelTmpIndi_flg_Inproc/1  "VTPM_RFWheelTmpIndi_flg"
  VTPM_RFWheelTmpIndi_flg_Inproc/1 -> UnitConverter420/1
  UnitConverter420/1 -> VOUTP_RFWheelTmpIndi_flg/1  "VOUTP_RFWheelTmpIndi_flg"
  VTPM_LRWheelTmpIndi_flg/1 -> VTPM_LRWheelTmpIndi_flg_Inproc/1  "VTPM_LRWheelTmpIndi_flg"
  VTPM_LRWheelTmpIndi_flg_Inproc/1 -> UnitConverter421/1
  UnitConverter421/1 -> VOUTP_LRWheelTmpIndi_flg/1  "VOUTP_LRWheelTmpIndi_flg"
  VTPM_RRWheelTmpIndi_flg/1 -> VTPM_RRWheelTmpIndi_flg_Inproc/1  "VTPM_RRWheelTmpIndi_flg"
  VTPM_RRWheelTmpIndi_flg_Inproc/1 -> UnitConverter422/1
  UnitConverter422/1 -> VOUTP_RRWheelTmpIndi_flg/1  "VOUTP_RRWheelTmpIndi_flg"
  VTPM_LFWheelPSW_raw8/1 -> VTPM_LFWheelPSW_raw8_Inproc/1  "VTPM_LFWheelPSW_raw8"
  VTPM_LFWheelPSW_raw8_Inproc/1 -> UnitConverter423/1
  UnitConverter423/1 -> VOUTP_LFWheelPSW_raw8/1  "VOUTP_LFWheelPSW_raw8"
  VTPM_LRWheelPSW_raw8/1 -> VTPM_LRWheelPSW_raw8_Inproc/1  "VTPM_LRWheelPSW_raw8"
  VTPM_LRWheelPSW_raw8_Inproc/1 -> UnitConverter424/1
  UnitConverter424/1 -> VOUTP_LRWheelPSW_raw8/1  "VOUTP_LRWheelPSW_raw8"
  VTPM_RFWheelPSW_raw8/1 -> VTPM_RFWheelPSW_raw8_Inproc/1  "VTPM_RFWheelPSW_raw8"
  VTPM_RFWheelPSW_raw8_Inproc/1 -> UnitConverter425/1
  UnitConverter425/1 -> VOUTP_RFWheelPSW_raw8/1  "VOUTP_RFWheelPSW_raw8"
  VTPM_RRWheelPSW_raw8/1 -> VTPM_RRWheelPSW_raw8_Inproc/1  "VTPM_RRWheelPSW_raw8"
  VTPM_RRWheelPSW_raw8_Inproc/1 -> UnitConverter426/1
  UnitConverter426/1 -> VOUTP_RRWheelPSW_raw8/1  "VOUTP_RRWheelPSW_raw8"
  VTPM_CWheelTips_enum/1 -> VTPM_CWheelTips_enum_Inproc/1  "VTPM_CWheelTips_enum"
  VTPM_CWheelTips_enum_Inproc/1 -> UnitConverter427/1
  UnitConverter427/1 -> VOUTP_CWheelTips_enum/1  "VOUTP_CWheelTips_enum"
  VTPM_AutoLTips_enum/1 -> VTPM_AutoLTips_enum_Inproc/1  "VTPM_AutoLTips_enum"
  VTPM_AutoLTips_enum_Inproc/1 -> UnitConverter428/1
  UnitConverter428/1 -> VOUTP_AutoLTips_enum/1  "VOUTP_AutoLTips_enum"
  VTPM_LFSensorMode_flg/1 -> VTPM_LFSensorMode_flg_Inproc/1  "VTPM_LFSensorMode_flg"
  VTPM_LFSensorMode_flg_Inproc/1 -> UnitConverter429/1
  UnitConverter429/1 -> VOUTP_LFSensorMode_flg/1  "VOUTP_LFSensorMode_flg"
  VTPM_RFSensorMode_flg/1 -> VTPM_RFSensorMode_flg_Inproc/1  "VTPM_RFSensorMode_flg"
  VTPM_RFSensorMode_flg_Inproc/1 -> UnitConverter430/1
  UnitConverter430/1 -> VOUTP_RFSensorMode_flg/1  "VOUTP_RFSensorMode_flg"
  VTPM_LRSensorMode_flg/1 -> VTPM_LRSensorMode_flg_Inproc/1  "VTPM_LRSensorMode_flg"
  VTPM_LRSensorMode_flg_Inproc/1 -> UnitConverter431/1
  UnitConverter431/1 -> VOUTP_LRSensorMode_flg/1  "VOUTP_LRSensorMode_flg"
  VTPM_RRSensorMode_flg/1 -> VTPM_RRSensorMode_flg_Inproc/1  "VTPM_RRSensorMode_flg"
  VTPM_RRSensorMode_flg_Inproc/1 -> UnitConverter432/1
  UnitConverter432/1 -> VOUTP_RRSensorMode_flg/1  "VOUTP_RRSensorMode_flg"
  VTPM_S1ID_raw32/1 -> VTPM_S1ID_raw32_Inproc/1  "VTPM_S1ID_raw32"
  VTPM_S1ID_raw32_Inproc/1 -> UnitConverter433/1
  UnitConverter433/1 -> VOUTP_S1ID_raw32/1  "VOUTP_S1ID_raw32"
  VTPM_S2ID_raw32/1 -> VTPM_S2ID_raw32_Inproc/1  "VTPM_S2ID_raw32"
  VTPM_S2ID_raw32_Inproc/1 -> UnitConverter434/1
  UnitConverter434/1 -> VOUTP_S2ID_raw32/1  "VOUTP_S2ID_raw32"
  VTPM_S3ID_raw32/1 -> VTPM_S3ID_raw32_Inproc/1  "VTPM_S3ID_raw32"
  VTPM_S3ID_raw32_Inproc/1 -> UnitConverter435/1
  UnitConverter435/1 -> VOUTP_S3ID_raw32/1  "VOUTP_S3ID_raw32"
  VTPM_S4ID_raw32/1 -> VTPM_S4ID_raw32_Inproc/1  "VTPM_S4ID_raw32"
  VTPM_S4ID_raw32_Inproc/1 -> UnitConverter436/1
  UnitConverter436/1 -> VOUTP_S4ID_raw32/1  "VOUTP_S4ID_raw32"
  VTPM_S1L_enum/1 -> VTPM_S1L_enum_Inproc/1  "VTPM_S1L_enum"
  VTPM_S1L_enum_Inproc/1 -> UnitConverter437/1
  UnitConverter437/1 -> VOUTP_S1L_enum/1  "VOUTP_S1L_enum"
  VTPM_S2L_enum/1 -> VTPM_S2L_enum_Inproc/1  "VTPM_S2L_enum"
  VTPM_S2L_enum_Inproc/1 -> UnitConverter438/1
  UnitConverter438/1 -> VOUTP_S2L_enum/1  "VOUTP_S2L_enum"
  VTPM_S3L_enum/1 -> VTPM_S3L_enum_Inproc/1  "VTPM_S3L_enum"
  VTPM_S3L_enum_Inproc/1 -> UnitConverter439/1
  UnitConverter439/1 -> VOUTP_S3L_enum/1  "VOUTP_S3L_enum"
  VTPM_S4L_enum/1 -> VTPM_S4L_enum_Inproc/1  "VTPM_S4L_enum"
  VTPM_S4L_enum_Inproc/1 -> UnitConverter440/1
  UnitConverter440/1 -> VOUTP_S4L_enum/1  "VOUTP_S4L_enum"
  VTPM_ALFin_flg/1 -> VTPM_ALFin_flg_Inproc/1  "VTPM_ALFin_flg"
  VTPM_ALFin_flg_Inproc/1 -> UnitConverter441/1
  UnitConverter441/1 -> VOUTP_ALFin_flg/1  "VOUTP_ALFin_flg"
  VTPM_LFP20_raw8/1 -> VTPM_LFP20_raw8_Inproc/1  "VTPM_LFP20_raw8"
  VTPM_LFP20_raw8_Inproc/1 -> UnitConverter442/1
  UnitConverter442/1 -> VOUTP_LFP20_raw8/1  "VOUTP_LFP20_raw8"
  VTPM_RFP20_raw8/1 -> VTPM_RFP20_raw8_Inproc/1  "VTPM_RFP20_raw8"
  VTPM_RFP20_raw8_Inproc/1 -> UnitConverter443/1
  UnitConverter443/1 -> VOUTP_RFP20_raw8/1  "VOUTP_RFP20_raw8"
  VTPM_LRP20_raw8/1 -> VTPM_LRP20_raw8_Inproc/1  "VTPM_LRP20_raw8"
  VTPM_LRP20_raw8_Inproc/1 -> UnitConverter444/1
  UnitConverter444/1 -> VOUTP_LRP20_raw8/1  "VOUTP_LRP20_raw8"
  VTPM_RRP20_raw8/1 -> VTPM_RRP20_raw8_Inproc/1  "VTPM_RRP20_raw8"
  VTPM_RRP20_raw8_Inproc/1 -> UnitConverter445/1
  UnitConverter445/1 -> VOUTP_RRP20_raw8/1  "VOUTP_RRP20_raw8"
  VTPM_FAT_flg/1 -> VTPM_FAT_flg_Inproc/1  "VTPM_FAT_flg"
  VTPM_FAT_flg_Inproc/1 -> UnitConverter446/1
  UnitConverter446/1 -> VOUTP_FAT_flg/1  "VOUTP_FAT_flg"
  VTPM_IDin_raw32/1 -> VTPM_IDin_raw32_Inproc/1  "VTPM_IDin_raw32"
  VTPM_IDin_raw32_Inproc/1 -> UnitConverter447/1
  UnitConverter447/1 -> VOUTP_IDin_raw32/1  "VOUTP_IDin_raw32"
  VTPM_S1WheelDebugALTU_pct/1 -> VTPM_S1WheelDebugALTU_pct_Inproc/1  "VTPM_S1WheelDebugALTU_pct"
  VTPM_S1WheelDebugALTU_pct_Inproc/1 -> UnitConverter448/1
  UnitConverter448/1 -> VOUTP_S1WheelDebugALTU_pct/1  "VOUTP_S1WheelDebugALTU_pct"
  VTPM_S2WheelDebugALTU_pct/1 -> VTPM_S2WheelDebugALTU_pct_Inproc/1  "VTPM_S2WheelDebugALTU_pct"
  VTPM_S2WheelDebugALTU_pct_Inproc/1 -> UnitConverter449/1
  UnitConverter449/1 -> VOUTP_S2WheelDebugALTU_pct/1  "VOUTP_S2WheelDebugALTU_pct"
  VTPM_S3WheelDebugALTU_pct/1 -> VTPM_S3WheelDebugALTU_pct_Inproc/1  "VTPM_S3WheelDebugALTU_pct"
  VTPM_S3WheelDebugALTU_pct_Inproc/1 -> UnitConverter450/1
  UnitConverter450/1 -> VOUTP_S3WheelDebugALTU_pct/1  "VOUTP_S3WheelDebugALTU_pct"
  VTPM_S4WheelDebugALTU_pct/1 -> VTPM_S4WheelDebugALTU_pct_Inproc/1  "VTPM_S4WheelDebugALTU_pct"
  VTPM_S4WheelDebugALTU_pct_Inproc/1 -> UnitConverter451/1
  UnitConverter451/1 -> VOUTP_S4WheelDebugALTU_pct/1  "VOUTP_S4WheelDebugALTU_pct"
  VTPM_ID1messageALTU_raw8/1 -> VTPM_ID1messageALTU_raw8_Inproc/1  "VTPM_ID1messageALTU_raw8"
  VTPM_ID1messageALTU_raw8_Inproc/1 -> UnitConverter452/1
  UnitConverter452/1 -> VOUTP_ID1messageALTU_raw8/1  "VOUTP_ID1messageALTU_raw8"
  VTPM_ID2messageALTU_raw8/1 -> VTPM_ID2messageALTU_raw8_Inproc/1  "VTPM_ID2messageALTU_raw8"
  VTPM_ID2messageALTU_raw8_Inproc/1 -> UnitConverter453/1
  UnitConverter453/1 -> VOUTP_ID2messageALTU_raw8/1  "VOUTP_ID2messageALTU_raw8"
  VTPM_ID3messageALTU_raw8/1 -> VTPM_ID3messageALTU_raw8_Inproc/1  "VTPM_ID3messageALTU_raw8"
  VTPM_ID3messageALTU_raw8_Inproc/1 -> UnitConverter454/1
  UnitConverter454/1 -> VOUTP_ID3messageALTU_raw8/1  "VOUTP_ID3messageALTU_raw8"
  VTPM_ID4messageALTU_raw8/1 -> VTPM_ID4messageALTU_raw8_Inproc/1  "VTPM_ID4messageALTU_raw8"
  VTPM_ID4messageALTU_raw8_Inproc/1 -> UnitConverter455/1
  UnitConverter455/1 -> VOUTP_ID4messageALTU_raw8/1  "VOUTP_ID4messageALTU_raw8"
  VTPM_Chkfin_flg/1 -> VTPM_Chkfin_flg_Inproc/1  "VTPM_Chkfin_flg"
  VTPM_Chkfin_flg_Inproc/1 -> UnitConverter456/1
  UnitConverter456/1 -> VOUTP_Chkfin_flg/1  "VOUTP_Chkfin_flg"
  VTPM_SetIDLoc_flg/1 -> VTPM_SetIDLoc_flg_Inproc/1  "VTPM_SetIDLoc_flg"
  VTPM_SetIDLoc_flg_Inproc/1 -> UnitConverter457/1
  UnitConverter457/1 -> VOUTP_SetIDLoc_flg/1  "VOUTP_SetIDLoc_flg"
  VTPM_TPMSStorge_flg/1 -> VTPM_TPMSStorge_flg_Inproc/1  "VTPM_TPMSStorge_flg"
  VTPM_TPMSStorge_flg_Inproc/1 -> UnitConverter458/1
  UnitConverter458/1 -> VOUTP_TPMSStorge_flg/1  "VOUTP_TPMSStorge_flg"
  VTPM_ChkStorge_flg/1 -> VTPM_ChkStorge_flg_Inproc/1  "VTPM_ChkStorge_flg"
  VTPM_ChkStorge_flg_Inproc/1 -> UnitConverter459/1
  UnitConverter459/1 -> VOUTP_ChkStorge_flg/1  "VOUTP_ChkStorge_flg"
  VTPM_TPMSResButt_flg/1 -> VTPM_TPMSResButt_flg_Inproc/1  "VTPM_TPMSResButt_flg"
  VTPM_TPMSResButt_flg_Inproc/1 -> UnitConverter460/1
  UnitConverter460/1 -> VOUTP_TPMSResButt_flg/1  "VOUTP_TPMSResButt_flg"
  VTPM_LFPindi_enum/1 -> VTPM_LFPindi_enum_Inproc/1  "VTPM_LFPindi_enum"
  VTPM_LFPindi_enum_Inproc/1 -> UnitConverter461/1
  UnitConverter461/1 -> VOUTP_LFPindi_enum/1  "VOUTP_LFPindi_enum"
  VTPM_RFPind_enum/1 -> VTPM_RFPind_enum_Inproc/1  "VTPM_RFPind_enum"
  VTPM_RFPind_enum_Inproc/1 -> UnitConverter462/1
  UnitConverter462/1 -> VOUTP_RFPind_enum/1  "VOUTP_RFPind_enum"
  VTPM_LRPindi_enum/1 -> VTPM_LRPindi_enum_Inproc/1  "VTPM_LRPindi_enum"
  VTPM_LRPindi_enum_Inproc/1 -> UnitConverter463/1
  UnitConverter463/1 -> VOUTP_LRPindi_enum/1  "VOUTP_LRPindi_enum"
  VTPM_RRPindi_enum/1 -> VTPM_RRPindi_enum_Inproc/1  "VTPM_RRPindi_enum"
  VTPM_RRPindi_enum_Inproc/1 -> UnitConverter464/1
  UnitConverter464/1 -> VOUTP_RRPindi_enum/1  "VOUTP_RRPindi_enum"
  VTPM_WriteChkLFID_raw/1 -> VTPM_WriteChkLFID_raw_Inproc/1  "VTPM_WriteChkLFID_raw"
  VTPM_WriteChkLFID_raw_Inproc/1 -> UnitConverter465/1
  UnitConverter465/1 -> VOUTP_WriteChkLFID_raw/1  "VOUTP_WriteChkLFID_raw"
  VTPM_WriteChkRFID_raw/1 -> VTPM_WriteChkRFID_raw_Inproc/1  "VTPM_WriteChkRFID_raw"
  VTPM_WriteChkRFID_raw_Inproc/1 -> UnitConverter466/1
  UnitConverter466/1 -> VOUTP_WriteChkRFID_raw/1  "VOUTP_WriteChkRFID_raw"
  VTPM_WriteChkLRID_raw/1 -> VTPM_WriteChkLRID_raw_Inproc/1  "VTPM_WriteChkLRID_raw"
  VTPM_WriteChkLRID_raw_Inproc/1 -> UnitConverter467/1
  UnitConverter467/1 -> VOUTP_WriteChkLRID_raw/1  "VOUTP_WriteChkLRID_raw"
  VTPM_WriteChkRRID_raw/1 -> VTPM_WriteChkRRID_raw_Inproc/1  "VTPM_WriteChkRRID_raw"
  VTPM_WriteChkRRID_raw_Inproc/1 -> UnitConverter468/1
  UnitConverter468/1 -> VOUTP_WriteChkRRID_raw/1  "VOUTP_WriteChkRRID_raw"
  VTPM_WriteChkfinLFID_raw/1 -> VTPM_WriteChkfinLFID_raw_Inproc/1  "VTPM_WriteChkfinLFID_raw"
  VTPM_WriteChkfinLFID_raw_Inproc/1 -> UnitConverter469/1
  UnitConverter469/1 -> VOUTP_WriteChkfinLFID_raw/1  "VOUTP_WriteChkfinLFID_raw"
  VTPM_WriteChkfinRFID_raw/1 -> VTPM_WriteChkfinRFID_raw_Inproc/1  "VTPM_WriteChkfinRFID_raw"
  VTPM_WriteChkfinRFID_raw_Inproc/1 -> UnitConverter470/1
  UnitConverter470/1 -> VOUTP_WriteChkfinRFID_raw/1  "VOUTP_WriteChkfinRFID_raw"
  VTPM_WriteChkfinLRID_raw/1 -> VTPM_WriteChkfinLRID_raw_Inproc/1  "VTPM_WriteChkfinLRID_raw"
  VTPM_WriteChkfinLRID_raw_Inproc/1 -> UnitConverter471/1
  UnitConverter471/1 -> VOUTP_WriteChkfinLRID_raw/1  "VOUTP_WriteChkfinLRID_raw"
  VTPM_WriteChkfinRRID_raw/1 -> VTPM_WriteChkfinRRID_raw_Inproc/1  "VTPM_WriteChkfinRRID_raw"
  VTPM_WriteChkfinRRID_raw_Inproc/1 -> UnitConverter472/1
  UnitConverter472/1 -> VOUTP_WriteChkfinRRID_raw/1  "VOUTP_WriteChkfinRRID_raw"
  VTPM_Flashchkdatavalid_enum/1 -> VTPM_Flashchkdatavalid_enum_Inproc/1  "VTPM_Flashchkdatavalid_enum"
  VTPM_Flashchkdatavalid_enum_Inproc/1 -> UnitConverter473/1
  UnitConverter473/1 -> VOUTP_Flashchkdatavalid_enum/1  "VOUTP_Flashchkdatavalid_enum"
  VTPM_Flashdatavalid_enum/1 -> VTPM_Flashdatavalid_enum_Inproc/1  "VTPM_Flashdatavalid_enum"
  VTPM_Flashdatavalid_enum_Inproc/1 -> UnitConverter474/1
  UnitConverter474/1 -> VOUTP_Flashdatavalid_enum/1  "VOUTP_Flashdatavalid_enum"
  VTPM_unlearnSfali_flg/1 -> VTPM_unlearnSfali_flg_Inproc/1  "VTPM_unlearnSfali_flg"
  VTPM_unlearnSfali_flg_Inproc/1 -> UnitConverter475/1
  UnitConverter475/1 -> VOUTP_unlearnSfali_flg/1  "VOUTP_unlearnSfali_flg"
  VTPM_unlearnSfailvalid_enum/1 -> VTPM_unlearnSfailvalid_enum_Inproc/1  "VTPM_unlearnSfailvalid_enum"
  VTPM_unlearnSfailvalid_enum_Inproc/1 -> UnitConverter476/1
  UnitConverter476/1 -> VOUTP_unlearnSfailvalid_enum/1  "VOUTP_unlearnSfailvalid_enum"
  VTPM_Prepresstempvalid_enum/1 -> VTPM_Prepresstempvalid_enum_Inproc/1  "VTPM_Prepresstempvalid_enum"
  VTPM_Prepresstempvalid_enum_Inproc/1 -> UnitConverter477/1
  UnitConverter477/1 -> VOUTP_Prepresstempvalid_enum/1  "VOUTP_Prepresstempvalid_enum"
  VTPM_FlashS1ID_raw/1 -> VTPM_FlashS1ID_raw_Inproc/1  "VTPM_FlashS1ID_raw"
  VTPM_FlashS1ID_raw_Inproc/1 -> UnitConverter478/1
  UnitConverter478/1 -> VOUTP_FlashS1ID_raw/1  "VOUTP_FlashS1ID_raw"
  VTPM_FlashS2ID_raw/1 -> VTPM_FlashS2ID_raw_Inproc/1  "VTPM_FlashS2ID_raw"
  VTPM_FlashS2ID_raw_Inproc/1 -> UnitConverter479/1
  UnitConverter479/1 -> VOUTP_FlashS2ID_raw/1  "VOUTP_FlashS2ID_raw"
  VTPM_FlashS3ID_raw/1 -> VTPM_FlashS3ID_raw_Inproc/1  "VTPM_FlashS3ID_raw"
  VTPM_FlashS3ID_raw_Inproc/1 -> UnitConverter480/1
  UnitConverter480/1 -> VOUTP_FlashS3ID_raw/1  "VOUTP_FlashS3ID_raw"
  VTPM_FlashS4ID_raw/1 -> VTPM_FlashS4ID_raw_Inproc/1  "VTPM_FlashS4ID_raw"
  VTPM_FlashS4ID_raw_Inproc/1 -> UnitConverter481/1
  UnitConverter481/1 -> VOUTP_FlashS4ID_raw/1  "VOUTP_FlashS4ID_raw"
  VTPM_FlashIDvalid_enum/1 -> VTPM_FlashIDvalid_enum_Inproc/1  "VTPM_FlashIDvalid_enum"
  VTPM_FlashIDvalid_enum_Inproc/1 -> UnitConverter482/1
  UnitConverter482/1 -> VOUTP_FlashIDvalid_enum/1  "VOUTP_FlashIDvalid_enum"
  VTQD_ParkRequest_flg/1 -> VTQD_ParkRequest_flg_Inproc/1  "VTQD_ParkRequest_flg"
  VTQD_ParkRequest_flg_Inproc/1 -> UnitConverter483/1
  UnitConverter483/1 -> VOUTP_ParkRequest_flg/1  "VOUTP_ParkRequest_flg"
  VTQD_TqSourceFr_enum/1 -> VTQD_TqSourceFr_enum_Inproc/1  "VTQD_TqSourceFr_enum"
  VTQD_TqSourceFr_enum_Inproc/1 -> UnitConverter484/1
  UnitConverter484/1 -> VOUTP_TqSourceFr_enum/1  "VOUTP_TqSourceFr_enum"
  VTQD_TqSourceRr_enum/1 -> VTQD_TqSourceRr_enum_Inproc/1  "VTQD_TqSourceRr_enum"
  VTQD_TqSourceRr_enum_Inproc/1 -> UnitConverter485/1
  UnitConverter485/1 -> VOUTP_TqSourceRr_enum/1  "VOUTP_TqSourceRr_enum"
  VTQD_FrEDUAvailBrkRgnTq_Nm/1 -> VTQD_FrEDUAvailBrkRgnTq_Nm_Inproc/1  "VTQD_FrEDUAvailBrkRgnTq_Nm"
  VTQD_FrEDUAvailBrkRgnTq_Nm_Inproc/1 -> UnitConverter486/1
  UnitConverter486/1 -> VOUTP_FrEDUAvailBrkRgnTq_Nm/1  "VOUTP_FrEDUAvailBrkRgnTq_Nm"
  VTQD_RrEDUAvailBrkRgnTq_Nm/1 -> VTQD_RrEDUAvailBrkRgnTq_Nm_Inproc/1  "VTQD_RrEDUAvailBrkRgnTq_Nm"
  VTQD_RrEDUAvailBrkRgnTq_Nm_Inproc/1 -> UnitConverter487/1
  UnitConverter487/1 -> VOUTP_RrEDUAvailBrkRgnTq_Nm/1  "VOUTP_RrEDUAvailBrkRgnTq_Nm"
  VTQD_EVDriveMode_enum/1 -> VTQD_EVDriveMode_enum_Inproc/1  "VTQD_EVDriveMode_enum"
  VTQD_EVDriveMode_enum_Inproc/1 -> UnitConverter488/1
  UnitConverter488/1 -> VOUTP_EVDriveMode_enum/1  "VOUTP_EVDriveMode_enum"
  VTQD_ShiftGearPosn_enum/1 -> VTQD_ShiftGearPosn_enum_Inproc/1  "VTQD_ShiftGearPosn_enum"
  VTQD_ShiftGearPosn_enum_Inproc/1 -> UnitConverter489/1
  UnitConverter489/1 -> VOUTP_ShiftGearPosn_enum/1  "VOUTP_ShiftGearPosn_enum"
  VTQD_PButtonSta_enum/1 -> VTQD_PButtonSta_enum_Inproc/1  "VTQD_PButtonSta_enum"
  VTQD_PButtonSta_enum_Inproc/1 -> UnitConverter490/1
  UnitConverter490/1 -> VOUTP_PButtonSta_enum/1  "VOUTP_PButtonSta_enum"
  VTQD_FrActvDmpDisabReq_flg/1 -> VTQD_FrActvDmpDisabReq_flg_Inproc/1  "VTQD_FrActvDmpDisabReq_flg"
  VTQD_FrActvDmpDisabReq_flg_Inproc/1 -> UnitConverter491/1
  UnitConverter491/1 -> VOUTP_FrActvDmpDisabReq_flg/1  "VOUTP_FrActvDmpDisabReq_flg"
  VTQD_RrActvDmpDisabReq_flg/1 -> VTQD_RrActvDmpDisabReq_flg_Inproc/1  "VTQD_RrActvDmpDisabReq_flg"
  VTQD_RrActvDmpDisabReq_flg_Inproc/1 -> UnitConverter492/1
  UnitConverter492/1 -> VOUTP_RrActvDmpDisabReq_flg/1  "VOUTP_RrActvDmpDisabReq_flg"
  VTQD_FrRgnDecrSta_flg/1 -> VTQD_FrRgnDecrSta_flg_Inproc/1  "VTQD_FrRgnDecrSta_flg"
  VTQD_FrRgnDecrSta_flg_Inproc/1 -> UnitConverter493/1
  UnitConverter493/1 -> VOUTP_FrRgnDecrSta_flg/1  "VOUTP_FrRgnDecrSta_flg"
  VTQD_RrRgnDecrSta_flg/1 -> VTQD_RrRgnDecrSta_flg_Inproc/1  "VTQD_RrRgnDecrSta_flg"
  VTQD_RrRgnDecrSta_flg_Inproc/1 -> UnitConverter494/1
  UnitConverter494/1 -> VOUTP_RrRgnDecrSta_flg/1  "VOUTP_RrRgnDecrSta_flg"
  VTQD_DriverWhlTqDemFr_Nm/1 -> VTQD_DriverWhlTqDemFr_Nm_Inproc/1  "VTQD_DriverWhlTqDemFr_Nm"
  VTQD_DriverWhlTqDemFr_Nm_Inproc/1 -> UnitConverter495/1
  UnitConverter495/1 -> VOUTP_DriverWhlTqDemFr_Nm/1  "VOUTP_DriverWhlTqDemFr_Nm"
  VTQD_DriverWhlTqDemRr_Nm/1 -> VTQD_DriverWhlTqDemRr_Nm_Inproc/1  "VTQD_DriverWhlTqDemRr_Nm"
  VTQD_DriverWhlTqDemRr_Nm_Inproc/1 -> UnitConverter496/1
  UnitConverter496/1 -> VOUTP_DriverWhlTqDemRr_Nm/1  "VOUTP_DriverWhlTqDemRr_Nm"
  VTQD_FrEDUActTq_Nm/1 -> VTQD_FrEDUActTq_Nm_Inproc/1  "VTQD_FrEDUActTq_Nm"
  VTQD_FrEDUActTq_Nm_Inproc/1 -> UnitConverter497/1
  UnitConverter497/1 -> VOUTP_FrEDUActTq_Nm/1  "VOUTP_FrEDUActTq_Nm"
  VTQD_RrEDUActTq_Nm/1 -> VTQD_RrEDUActTq_Nm_Inproc/1  "VTQD_RrEDUActTq_Nm"
  VTQD_RrEDUActTq_Nm_Inproc/1 -> UnitConverter498/1
  UnitConverter498/1 -> VOUTP_RrEDUActTq_Nm/1  "VOUTP_RrEDUActTq_Nm"
  VTQD_FrEDURolRgnTq_Nm/1 -> VTQD_FrEDURolRgnTq_Nm_Inproc/1  "VTQD_FrEDURolRgnTq_Nm"
  VTQD_FrEDURolRgnTq_Nm_Inproc/1 -> UnitConverter499/1
  UnitConverter499/1 -> VOUTP_FrEDURolRgnTq_Nm/1  "VOUTP_FrEDURolRgnTq_Nm"
  VTQD_RrEDURolRgnTq_Nm/1 -> VTQD_RrEDURolRgnTq_Nm_Inproc/1  "VTQD_RrEDURolRgnTq_Nm"
  VTQD_RrEDURolRgnTq_Nm_Inproc/1 -> UnitConverter500/1
  UnitConverter500/1 -> VOUTP_RrEDURolRgnTq_Nm/1  "VOUTP_RrEDURolRgnTq_Nm"
  VTQD_FrEDUSpd_rpm/1 -> VTQD_FrEDUSpd_rpm_Inproc/1  "VTQD_FrEDUSpd_rpm"
  VTQD_FrEDUSpd_rpm_Inproc/1 -> UnitConverter501/1
  UnitConverter501/1 -> VOUTP_FrEDUSpd_rpm/1  "VOUTP_FrEDUSpd_rpm"
  VTQD_RrEDUSpd_rpm/1 -> VTQD_RrEDUSpd_rpm_Inproc/1  "VTQD_RrEDUSpd_rpm"
  VTQD_RrEDUSpd_rpm_Inproc/1 -> UnitConverter502/1
  UnitConverter502/1 -> VOUTP_RrEDUSpd_rpm/1  "VOUTP_RrEDUSpd_rpm"
  VTQD_FrEDUSpdValid_flg/1 -> VTQD_FrEDUSpdValid_flg_Inproc/1  "VTQD_FrEDUSpdValid_flg"
  VTQD_FrEDUSpdValid_flg_Inproc/1 -> UnitConverter503/1
  UnitConverter503/1 -> VOUTP_FrEDUSpdValid_flg/1  "VOUTP_FrEDUSpdValid_flg"
  VTQD_FrEDUAvailBrkRgnTqV_flg/1 -> VTQD_FrEDUAvailBrkRgnTqV_flg_Inproc/1  "VTQD_FrEDUAvailBrkRgnTqV_flg"
  VTQD_FrEDUAvailBrkRgnTqV_flg_Inproc/1 -> UnitConverter504/1
  UnitConverter504/1 -> VOUTP_FrEDUAvailBrkRgnTqV_flg/1  "VOUTP_FrEDUAvailBrkRgnTqV_flg"
  VTQD_RrEDUSpdValid_flg/1 -> VTQD_RrEDUSpdValid_flg_Inproc/1  "VTQD_RrEDUSpdValid_flg"
  VTQD_RrEDUSpdValid_flg_Inproc/1 -> UnitConverter505/1
  UnitConverter505/1 -> VOUTP_RrEDUSpdValid_flg/1  "VOUTP_RrEDUSpdValid_flg"
  VTQD_RrEDUAvailBrkRgnTqV_flg/1 -> VTQD_RrEDUAvailBrkRgnTqV_flg_Inproc/1  "VTQD_RrEDUAvailBrkRgnTqV_flg"
  VTQD_RrEDUAvailBrkRgnTqV_flg_Inproc/1 -> UnitConverter506/1
  UnitConverter506/1 -> VOUTP_RrEDUAvailBrkRgnTqV_flg/1  "VOUTP_RrEDUAvailBrkRgnTqV_flg"
  VTQD_RgnAbnorSta_flg/1 -> VTQD_RgnAbnorSta_flg_Inproc/1  "VTQD_RgnAbnorSta_flg"
  VTQD_RgnAbnorSta_flg_Inproc/1 -> UnitConverter507/1
  UnitConverter507/1 -> VOUTP_RgnAbnorSta_flg/1  "VOUTP_RgnAbnorSta_flg"
  VTQD_PTCSPermSta_flg/1 -> VTQD_PTCSPermSta_flg_Inproc/1  "VTQD_PTCSPermSta_flg"
  VTQD_PTCSPermSta_flg_Inproc/1 -> UnitConverter508/1
  UnitConverter508/1 -> VOUTP_PTCSPermSta_flg/1  "VOUTP_PTCSPermSta_flg"
  VTQD_FrRgnPermSta_flg/1 -> VTQD_FrRgnPermSta_flg_Inproc/1  "VTQD_FrRgnPermSta_flg"
  VTQD_FrRgnPermSta_flg_Inproc/1 -> UnitConverter509/1
  UnitConverter509/1 -> VOUTP_FrRgnPermSta_flg/1  "VOUTP_FrRgnPermSta_flg"
  VTQD_RrRgnPermSta_flg/1 -> VTQD_RrRgnPermSta_flg_Inproc/1  "VTQD_RrRgnPermSta_flg"
  VTQD_RrRgnPermSta_flg_Inproc/1 -> UnitConverter510/1
  UnitConverter510/1 -> VOUTP_RrRgnPermSta_flg/1  "VOUTP_RrRgnPermSta_flg"
  VTQD_FrIdcMin_A/1 -> VTQD_FrIdcMin_A_Inproc/1  "VTQD_FrIdcMin_A"
  VTQD_FrIdcMin_A_Inproc/1 -> UnitConverter511/1
  UnitConverter511/1 -> VOUTP_FrIdcMin_A/1  "VOUTP_FrIdcMin_A"
  VTQD_FrIdcMax_A/1 -> VTQD_FrIdcMax_A_Inproc/1  "VTQD_FrIdcMax_A"
  VTQD_FrIdcMax_A_Inproc/1 -> UnitConverter512/1
  UnitConverter512/1 -> VOUTP_FrIdcMax_A/1  "VOUTP_FrIdcMax_A"
  VTQD_FrUdcMin_V/1 -> VTQD_FrUdcMin_V_Inproc/1  "VTQD_FrUdcMin_V"
  VTQD_FrUdcMin_V_Inproc/1 -> UnitConverter513/1
  UnitConverter513/1 -> VOUTP_FrUdcMin_V/1  "VOUTP_FrUdcMin_V"
  VTQD_FrUdcMax_V/1 -> VTQD_FrUdcMax_V_Inproc/1  "VTQD_FrUdcMax_V"
  VTQD_FrUdcMax_V_Inproc/1 -> UnitConverter514/1
  UnitConverter514/1 -> VOUTP_FrUdcMax_V/1  "VOUTP_FrUdcMax_V"
  VTQD_RrIdcMin_A/1 -> VTQD_RrIdcMin_A_Inproc/1  "VTQD_RrIdcMin_A"
  VTQD_RrIdcMin_A_Inproc/1 -> UnitConverter515/1
  UnitConverter515/1 -> VOUTP_RrIdcMin_A/1  "VOUTP_RrIdcMin_A"
  VTQD_RrIdcMax_A/1 -> VTQD_RrIdcMax_A_Inproc/1  "VTQD_RrIdcMax_A"
  VTQD_RrIdcMax_A_Inproc/1 -> UnitConverter516/1
  UnitConverter516/1 -> VOUTP_RrIdcMax_A/1  "VOUTP_RrIdcMax_A"
  VTQD_RrUdcMin_V/1 -> VTQD_RrUdcMin_V_Inproc/1  "VTQD_RrUdcMin_V"
  VTQD_RrUdcMin_V_Inproc/1 -> UnitConverter517/1
  UnitConverter517/1 -> VOUTP_RrUdcMin_V/1  "VOUTP_RrUdcMin_V"
  VTQD_RrUdcMax_V/1 -> VTQD_RrUdcMax_V_Inproc/1  "VTQD_RrUdcMax_V"
  VTQD_RrUdcMax_V_Inproc/1 -> UnitConverter518/1
  UnitConverter518/1 -> VOUTP_RrUdcMax_V/1  "VOUTP_RrUdcMax_V"
  VTQD_ReBrakeLPReq_flg/1 -> VTQD_ReBrakeLPReq_flg_Inproc/1  "VTQD_ReBrakeLPReq_flg"
  VTQD_ReBrakeLPReq_flg_Inproc/1 -> UnitConverter519/1
  UnitConverter519/1 -> VOUTP_ReBrakeLPReq_flg/1  "VOUTP_ReBrakeLPReq_flg"
  VTQD_CreepON_flg/1 -> VTQD_CreepON_flg_Inproc/1  "VTQD_CreepON_flg"
  VTQD_CreepON_flg_Inproc/1 -> UnitConverter520/1
  UnitConverter520/1 -> VOUTP_CreepON_flg/1  "VOUTP_CreepON_flg"
  VTQD_ActEMpTrq_pct/1 -> VTQD_ActEMpTrq_pct_Inproc/1  "VTQD_ActEMpTrq_pct"
  VTQD_ActEMpTrq_pct_Inproc/1 -> UnitConverter521/1
  UnitConverter521/1 -> VOUTP_ActEMpTrq_pct/1  "VOUTP_ActEMpTrq_pct"
  VTQD_ActMaxAvaEMRecpTrq_pct/1 -> VTQD_ActMaxAvaEMRecpTrq_pct_Inproc/1  "VTQD_ActMaxAvaEMRecpTrq_pct"
  VTQD_ActMaxAvaEMRecpTrq_pct_Inproc/1 -> UnitConverter522/1
  UnitConverter522/1 -> VOUTP_ActMaxAvaEMRecpTrq_pct/1  "VOUTP_ActMaxAvaEMRecpTrq_pct"
  VTQD_ActDriveDirect_enum/1 -> VTQD_ActDriveDirect_enum_Inproc/1  "VTQD_ActDriveDirect_enum"
  VTQD_ActDriveDirect_enum_Inproc/1 -> UnitConverter523/1
  UnitConverter523/1 -> VOUTP_ActDriveDirect_enum/1  "VOUTP_ActDriveDirect_enum"
  VTQD_DLEngaged_enum/1 -> VTQD_DLEngaged_enum_Inproc/1  "VTQD_DLEngaged_enum"
  VTQD_DLEngaged_enum_Inproc/1 -> UnitConverter524/1
  UnitConverter524/1 -> VOUTP_DLEngaged_enum/1  "VOUTP_DLEngaged_enum"
  VTQD_EMTrqModeDrvBrk_enum/1 -> VTQD_EMTrqModeDrvBrk_enum_Inproc/1  "VTQD_EMTrqModeDrvBrk_enum"
  VTQD_EMTrqModeDrvBrk_enum_Inproc/1 -> UnitConverter525/1
  UnitConverter525/1 -> VOUTP_EMTrqModeDrvBrk_enum/1  "VOUTP_EMTrqModeDrvBrk_enum"
  VTQD_ActEMpTrqHrls_pct/1 -> VTQD_ActEMpTrqHrls_pct_Inproc/1  "VTQD_ActEMpTrqHrls_pct"
  VTQD_ActEMpTrqHrls_pct_Inproc/1 -> UnitConverter526/1
  UnitConverter526/1 -> VOUTP_ActEMpTrqHrls_pct/1  "VOUTP_ActEMpTrqHrls_pct"
  VTQD_ActEMOutSftSpd_rpm/1 -> VTQD_ActEMOutSftSpd_rpm_Inproc/1  "VTQD_ActEMOutSftSpd_rpm"
  VTQD_ActEMOutSftSpd_rpm_Inproc/1 -> UnitConverter527/1
  UnitConverter527/1 -> VOUTP_ActEMOutSftSpd_rpm/1  "VOUTP_ActEMOutSftSpd_rpm"
  VTQD_DrvDemEMRtapTrq_pct/1 -> VTQD_DrvDemEMRtapTrq_pct_Inproc/1  "VTQD_DrvDemEMRtapTrq_pct"
  VTQD_DrvDemEMRtapTrq_pct_Inproc/1 -> UnitConverter528/1
  UnitConverter528/1 -> VOUTP_DrvDemEMRtapTrq_pct/1  "VOUTP_DrvDemEMRtapTrq_pct"
  VTQD_SACtrlDev_enum/1 -> VTQD_SACtrlDev_enum_Inproc/1  "VTQD_SACtrlDev_enum"
  VTQD_SACtrlDev_enum_Inproc/1 -> UnitConverter529/1
  UnitConverter529/1 -> VOUTP_SACtrlDev_enum/1  "VOUTP_SACtrlDev_enum"
  VTQD_RetSelNonEng_pct/1 -> VTQD_RetSelNonEng_pct_Inproc/1  "VTQD_RetSelNonEng_pct"
  VTQD_RetSelNonEng_pct_Inproc/1 -> UnitConverter530/1
  UnitConverter530/1 -> VOUTP_RetSelNonEng_pct/1  "VOUTP_RetSelNonEng_pct"
  VTQD_ShiftPgs_enum/1 -> VTQD_ShiftPgs_enum_Inproc/1  "VTQD_ShiftPgs_enum"
  VTQD_ShiftPgs_enum_Inproc/1 -> UnitConverter531/1
  UnitConverter531/1 -> VOUTP_ShiftPgs_enum/1  "VOUTP_ShiftPgs_enum"
  VTQD_AccPedal1LowSW_enum/1 -> VTQD_AccPedal1LowSW_enum_Inproc/1  "VTQD_AccPedal1LowSW_enum"
  VTQD_AccPedal1LowSW_enum_Inproc/1 -> UnitConverter532/1
  UnitConverter532/1 -> VOUTP_AccPedal1LowSW_enum/1  "VOUTP_AccPedal1LowSW_enum"
  VTQD_AccPedalPos1_pct/1 -> VTQD_AccPedalPos1_pct_Inproc/1  "VTQD_AccPedalPos1_pct"
  VTQD_AccPedalPos1_pct_Inproc/1 -> UnitConverter533/1
  UnitConverter533/1 -> VOUTP_AccPedalPos1_pct/1  "VOUTP_AccPedalPos1_pct"
  VTQD_ParkBrakeSW_enum/1 -> VTQD_ParkBrakeSW_enum_Inproc/1  "VTQD_ParkBrakeSW_enum"
  VTQD_ParkBrakeSW_enum_Inproc/1 -> UnitConverter534/1
  UnitConverter534/1 -> VOUTP_ParkBrakeSW_enum/1  "VOUTP_ParkBrakeSW_enum"
  VTQD_VCUVehSpd_kph/1 -> VTQD_VCUVehSpd_kph_Inproc/1  "VTQD_VCUVehSpd_kph"
  VTQD_VCUVehSpd_kph_Inproc/1 -> UnitConverter535/1
  UnitConverter535/1 -> VOUTP_VCUVehSpd_kph/1  "VOUTP_VCUVehSpd_kph"
  VTQD_BrakeSW_enum/1 -> VTQD_BrakeSW_enum_Inproc/1  "VTQD_BrakeSW_enum"
  VTQD_BrakeSW_enum_Inproc/1 -> UnitConverter536/1
  UnitConverter536/1 -> VOUTP_BrakeSW_enum/1  "VOUTP_BrakeSW_enum"
  VTQD_NFricPercTorq_pct/1 -> VTQD_NFricPercTorq_pct_Inproc/1  "VTQD_NFricPercTorq_pct"
  VTQD_NFricPercTorq_pct_Inproc/1 -> UnitConverter537/1
  UnitConverter537/1 -> VOUTP_NFricPercTorq_pct/1  "VOUTP_NFricPercTorq_pct"
  VTQD_EMParasLoss_pct/1 -> VTQD_EMParasLoss_pct_Inproc/1  "VTQD_EMParasLoss_pct"
  VTQD_EMParasLoss_pct_Inproc/1 -> UnitConverter538/1
  UnitConverter538/1 -> VOUTP_EMParasLoss_pct/1  "VOUTP_EMParasLoss_pct"
  VTQD_EEC2MSGCnt_raw/1 -> VTQD_EEC2MSGCnt_raw_Inproc/1  "VTQD_EEC2MSGCnt_raw"
  VTQD_EEC2MSGCnt_raw_Inproc/1 -> UnitConverter539/1
  UnitConverter539/1 -> VOUTP_EEC2MSGCnt_raw/1  "VOUTP_EEC2MSGCnt_raw"
  VTQD_EEC2MSGCS_raw/1 -> VTQD_EEC2MSGCS_raw_Inproc/1  "VTQD_EEC2MSGCS_raw"
  VTQD_EEC2MSGCS_raw_Inproc/1 -> UnitConverter540/1
  UnitConverter540/1 -> VOUTP_EEC2MSGCS_raw/1  "VOUTP_EEC2MSGCS_raw"
  VTQD_FDCCHAEBSRd4BRSta_enum/1 -> VTQD_FDCCHAEBSRd4BRSta_enum_Inproc/1  "VTQD_FDCCHAEBSRd4BRSta_enum"
  VTQD_FDCCHAEBSRd4BRSta_enum_Inproc/1 -> UnitConverter541/1
  UnitConverter541/1 -> VOUTP_FDCCHAEBSRd4BRSta_enum/1  "VOUTP_FDCCHAEBSRd4BRSta_enum"
  VTQD_FDCCHAEBSHBSwSta_enum/1 -> VTQD_FDCCHAEBSHBSwSta_enum_Inproc/1  "VTQD_FDCCHAEBSHBSwSta_enum"
  VTQD_FDCCHAEBSHBSwSta_enum_Inproc/1 -> UnitConverter542/1
  UnitConverter542/1 -> VOUTP_FDCCHAEBSHBSwSta_enum/1  "VOUTP_FDCCHAEBSHBSwSta_enum"
  VTQD_FDCCHAEBSHHSwSta_enum/1 -> VTQD_FDCCHAEBSHHSwSta_enum_Inproc/1  "VTQD_FDCCHAEBSHHSwSta_enum"
  VTQD_FDCCHAEBSHHSwSta_enum_Inproc/1 -> UnitConverter543/1
  UnitConverter543/1 -> VOUTP_FDCCHAEBSHHSwSta_enum/1  "VOUTP_FDCCHAEBSHHSwSta_enum"
  VTQD_FDCVCUTUpAStaSta_enum/1 -> VTQD_FDCVCUTUpAStaSta_enum_Inproc/1  "VTQD_FDCVCUTUpAStaSta_enum"
  VTQD_FDCVCUTUpAStaSta_enum_Inproc/1 -> UnitConverter544/1
  UnitConverter544/1 -> VOUTP_FDCVCUTUpAStaSta_enum/1  "VOUTP_FDCVCUTUpAStaSta_enum"
  VTQD_FDCVCUDACStatusSta_enum/1 -> VTQD_FDCVCUDACStatusSta_enum_Inproc/1  "VTQD_FDCVCUDACStatusSta_enum"
  VTQD_FDCVCUDACStatusSta_enum_Inproc/1 -> UnitConverter545/1
  UnitConverter545/1 -> VOUTP_FDCVCUDACStatusSta_enum/1  "VOUTP_FDCVCUDACStatusSta_enum"
  VTQR_FrTMTqReq_Nm/1 -> VTQR_FrTMTqReq_Nm_Inproc/1  "VTQR_FrTMTqReq_Nm"
  VTQR_FrTMTqReq_Nm_Inproc/1 -> UnitConverter546/1
  UnitConverter546/1 -> VOUTP_FrTMTqReq_Nm/1  "VOUTP_FrTMTqReq_Nm"
  VTQR_RrTMTqReq_Nm/1 -> VTQR_RrTMTqReq_Nm_Inproc/1  "VTQR_RrTMTqReq_Nm"
  VTQR_RrTMTqReq_Nm_Inproc/1 -> UnitConverter547/1
  UnitConverter547/1 -> VOUTP_RrTMTqReq_Nm/1  "VOUTP_RrTMTqReq_Nm"
  VV2L_ReqOBCV2LEna_enum/1 -> VV2L_ReqOBCV2LEna_enum_Inproc/1  "VV2L_ReqOBCV2LEna_enum"
  VV2L_ReqOBCV2LEna_enum_Inproc/1 -> UnitConverter548/1
  UnitConverter548/1 -> VOUTP_ReqOBCV2LEna_enum/1  "VOUTP_ReqOBCV2LEna_enum"
  VV2L_ReqV2LIVIPopup_enum/1 -> VV2L_ReqV2LIVIPopup_enum_Inproc/1  "VV2L_ReqV2LIVIPopup_enum"
  VV2L_ReqV2LIVIPopup_enum_Inproc/1 -> UnitConverter549/1
  UnitConverter549/1 -> VOUTP_ReqV2LIVIPopup_enum/1  "VOUTP_ReqV2LIVIPopup_enum"
  VVMC_FeatSetSpdFinal_raw32/1 -> VVMC_FeatSetSpdFinal_raw32_Inproc/1  "VVMC_FeatSetSpdFinal_raw32"
  VVMC_FeatSetSpdFinal_raw32_Inproc/1 -> UnitConverter550/1
  UnitConverter550/1 -> VOUTP_FeatSetSpdFinal_raw32/1  "VOUTP_FeatSetSpdFinal_raw32"
  VVMC_VehicleSpeed_mph/1 -> VVMC_VehicleSpeed_mph_Inproc/1  "VVMC_VehicleSpeed_mph"
  VVMC_VehicleSpeed_mph_Inproc/1 -> UnitConverter551/1
  UnitConverter551/1 -> VOUTP_VehicleSpeed_mph/1  "VOUTP_VehicleSpeed_mph"
  VVMC_VehicleSpeed_kph/1 -> VVMC_VehicleSpeed_kph_Inproc/1  "VVMC_VehicleSpeed_kph"
  VVMC_VehicleSpeed_kph_Inproc/1 -> UnitConverter552/1
  UnitConverter552/1 -> VOUTP_VehicleSpeed_kph/1  "VOUTP_VehicleSpeed_kph"
  VVMC_MeterIndSpeed_raw32/1 -> VVMC_MeterIndSpeed_raw32_Inproc/1  "VVMC_MeterIndSpeed_raw32"
  VVMC_MeterIndSpeed_raw32_Inproc/1 -> UnitConverter553/1
  UnitConverter553/1 -> VOUTP_MeterIndSpeed_raw32/1  "VOUTP_MeterIndSpeed_raw32"
  VVMC_VMCAEBCtrlAvail_flg/1 -> VVMC_VMCAEBCtrlAvail_flg_Inproc/1  "VVMC_VMCAEBCtrlAvail_flg"
  VVMC_VMCAEBCtrlAvail_flg_Inproc/1 -> UnitConverter554/1
  UnitConverter554/1 -> VOUTP_VMCAEBCtrlAvail_flg/1  "VOUTP_VMCAEBCtrlAvail_flg"
  VVMC_VMCACCCtrlAvail_flg/1 -> VVMC_VMCACCCtrlAvail_flg_Inproc/1  "VVMC_VMCACCCtrlAvail_flg"
  VVMC_VMCACCCtrlAvail_flg_Inproc/1 -> UnitConverter555/1
  UnitConverter555/1 -> VOUTP_VMCACCCtrlAvail_flg/1  "VOUTP_VMCACCCtrlAvail_flg"
  VVMC_VMCCCCtrlAvail_flg/1 -> VVMC_VMCCCCtrlAvail_flg_Inproc/1  "VVMC_VMCCCCtrlAvail_flg"
  VVMC_VMCCCCtrlAvail_flg_Inproc/1 -> UnitConverter556/1
  UnitConverter556/1 -> VOUTP_VMCCCCtrlAvail_flg/1  "VOUTP_VMCCCCtrlAvail_flg"
  VVMC_VMCMSACtrlAvail_flg/1 -> VVMC_VMCMSACtrlAvail_flg_Inproc/1  "VVMC_VMCMSACtrlAvail_flg"
  VVMC_VMCMSACtrlAvail_flg_Inproc/1 -> UnitConverter557/1
  UnitConverter557/1 -> VOUTP_VMCMSACtrlAvail_flg/1  "VOUTP_VMCMSACtrlAvail_flg"
  VVMC_FeatArbitrSta_enum/1 -> VVMC_FeatArbitrSta_enum_Inproc/1  "VVMC_FeatArbitrSta_enum"
  VVMC_FeatArbitrSta_enum_Inproc/1 -> UnitConverter558/1
  UnitConverter558/1 -> VOUTP_FeatArbitrSta_enum/1  "VOUTP_FeatArbitrSta_enum"
  VVMC_FeatReqSpd_kph/1 -> VVMC_FeatReqSpd_kph_Inproc/1  "VVMC_FeatReqSpd_kph"
  VVMC_FeatReqSpd_kph_Inproc/1 -> UnitConverter559/1
  UnitConverter559/1 -> VOUTP_FeatReqSpd_kph/1  "VOUTP_FeatReqSpd_kph"
  VVMC_JerkPCT_pct/1 -> VVMC_JerkPCT_pct_Inproc/1  "VVMC_JerkPCT_pct"
  VVMC_JerkPCT_pct_Inproc/1 -> UnitConverter560/1
  UnitConverter560/1 -> VOUTP_JerkPCT_pct/1  "VOUTP_JerkPCT_pct"
  VVMC_LimitPCT_pct/1 -> VVMC_LimitPCT_pct_Inproc/1  "VVMC_LimitPCT_pct"
  VVMC_LimitPCT_pct_Inproc/1 -> UnitConverter561/1
  UnitConverter561/1 -> VOUTP_LimitPCT_pct/1  "VOUTP_LimitPCT_pct"
  VVMC_FrontRearSlipRatioCtrl_flg/1 -> VVMC_FrontRearSlipRatioCtrl_flg_Inproc/1  "VVMC_FrontRearSlipRatioCtrl_flg"
  VVMC_FrontRearSlipRatioCtrl_flg_Inproc/1 -> UnitConverter562/1
  UnitConverter562/1 -> VOUTP_FrontRearSlipRatioCtrl_flg/1  "VOUTP_FrontRearSlipRatioCtrl_flg"
  VVMC_RearWhlSlipRatioCtrl_flg/1 -> VVMC_RearWhlSlipRatioCtrl_flg_Inproc/1  "VVMC_RearWhlSlipRatioCtrl_flg"
  VVMC_RearWhlSlipRatioCtrl_flg_Inproc/1 -> UnitConverter563/1
  UnitConverter563/1 -> VOUTP_RearWhlSlipRatioCtrl_flg/1  "VOUTP_RearWhlSlipRatioCtrl_flg"
  VVMC_SingleWhlSlipRatioCtrl_flg/1 -> VVMC_SingleWhlSlipRatioCtrl_flg_Inproc/1  "VVMC_SingleWhlSlipRatioCtrl_flg"
  VVMC_SingleWhlSlipRatioCtrl_flg_Inproc/1 -> UnitConverter564/1
  UnitConverter564/1 -> VOUTP_SingleWhlSlipRatioCtrl_flg/1  "VOUTP_SingleWhlSlipRatioCtrl_flg"
  VVMC_LatAccCtrl_flg/1 -> VVMC_LatAccCtrl_flg_Inproc/1  "VVMC_LatAccCtrl_flg"
  VVMC_LatAccCtrl_flg_Inproc/1 -> UnitConverter565/1
  UnitConverter565/1 -> VOUTP_LatAccCtrl_flg/1  "VOUTP_LatAccCtrl_flg"
  VVMC_SafetyCtrl_flg/1 -> VVMC_SafetyCtrl_flg_Inproc/1  "VVMC_SafetyCtrl_flg"
  VVMC_SafetyCtrl_flg_Inproc/1 -> UnitConverter566/1
  UnitConverter566/1 -> VOUTP_SafetyCtrl_flg/1  "VOUTP_SafetyCtrl_flg"
  VVMC_SPD2ACCAct_flg/1 -> VVMC_SPD2ACCAct_flg_Inproc/1  "VVMC_SPD2ACCAct_flg"
  VVMC_SPD2ACCAct_flg_Inproc/1 -> UnitConverter567/1
  UnitConverter567/1 -> VOUTP_SPD2ACCAct_flg/1  "VOUTP_SPD2ACCAct_flg"
  VVMC_AccCalcuPID_mps2/1 -> VVMC_AccCalcuPID_mps2_Inproc/1  "VVMC_AccCalcuPID_mps2"
  VVMC_AccCalcuPID_mps2_Inproc/1 -> UnitConverter568/1
  UnitConverter568/1 -> VOUTP_AccCalcuPID_mps2/1  "VOUTP_AccCalcuPID_mps2"
  VVMC_ISOAccLimit_mps2/1 -> VVMC_ISOAccLimit_mps2_Inproc/1  "VVMC_ISOAccLimit_mps2"
  VVMC_ISOAccLimit_mps2_Inproc/1 -> UnitConverter569/1
  UnitConverter569/1 -> VOUTP_ISOAccLimit_mps2/1  "VOUTP_ISOAccLimit_mps2"
  VVMC_ISODecLimit_mps2/1 -> VVMC_ISODecLimit_mps2_Inproc/1  "VVMC_ISODecLimit_mps2"
  VVMC_ISODecLimit_mps2_Inproc/1 -> UnitConverter570/1
  UnitConverter570/1 -> VOUTP_ISODecLimit_mps2/1  "VOUTP_ISODecLimit_mps2"
  VVMC_ISOJerkLimit_mps3/1 -> VVMC_ISOJerkLimit_mps3_Inproc/1  "VVMC_ISOJerkLimit_mps3"
  VVMC_ISOJerkLimit_mps3_Inproc/1 -> UnitConverter571/1
  UnitConverter571/1 -> VOUTP_ISOJerkLimit_mps3/1  "VOUTP_ISOJerkLimit_mps3"
  VVMC_ACCRequiredAccel_mps2/1 -> VVMC_ACCRequiredAccel_mps2_Inproc/1  "VVMC_ACCRequiredAccel_mps2"
  VVMC_ACCRequiredAccel_mps2_Inproc/1 -> UnitConverter572/1
  UnitConverter572/1 -> VOUTP_ACCRequiredAccel_mps2/1  "VOUTP_ACCRequiredAccel_mps2"
  VVMC_DISCReqAcc_mps2/1 -> VVMC_DISCReqAcc_mps2_Inproc/1  "VVMC_DISCReqAcc_mps2"
  VVMC_DISCReqAcc_mps2_Inproc/1 -> UnitConverter573/1
  UnitConverter573/1 -> VOUTP_DISCReqAcc_mps2/1  "VOUTP_DISCReqAcc_mps2"
  VVMC_FeatArbitrFinal_enum/1 -> VVMC_FeatArbitrFinal_enum_Inproc/1  "VVMC_FeatArbitrFinal_enum"
  VVMC_FeatArbitrFinal_enum_Inproc/1 -> UnitConverter574/1
  UnitConverter574/1 -> VOUTP_FeatArbitrFinal_enum/1  "VOUTP_FeatArbitrFinal_enum"
  VVMC_LateralCtrl_flg/1 -> VVMC_LateralCtrl_flg_Inproc/1  "VVMC_LateralCtrl_flg"
  VVMC_LateralCtrl_flg_Inproc/1 -> UnitConverter575/1
  UnitConverter575/1 -> VOUTP_LateralCtrl_flg/1  "VOUTP_LateralCtrl_flg"
  VVMC_ADASLKASta_enum/1 -> VVMC_ADASLKASta_enum_Inproc/1  "VVMC_ADASLKASta_enum"
  VVMC_ADASLKASta_enum_Inproc/1 -> UnitConverter576/1
  UnitConverter576/1 -> VOUTP_ADASLKASta_enum/1  "VOUTP_ADASLKASta_enum"
  VVMC_LKAStrToqReq_Nm/1 -> VVMC_LKAStrToqReq_Nm_Inproc/1  "VVMC_LKAStrToqReq_Nm"
  VVMC_LKAStrToqReq_Nm_Inproc/1 -> UnitConverter577/1
  UnitConverter577/1 -> VOUTP_LKAStrToqReq_Nm/1  "VOUTP_LKAStrToqReq_Nm"
  VVMC_LKATOIFault_flg/1 -> VVMC_LKATOIFault_flg_Inproc/1  "VVMC_LKATOIFault_flg"
  VVMC_LKATOIFault_flg_Inproc/1 -> UnitConverter578/1
  UnitConverter578/1 -> VOUTP_LKATOIFault_flg/1  "VOUTP_LKATOIFault_flg"
  VVMC_LKATOIAct_enum/1 -> VVMC_LKATOIAct_enum_Inproc/1  "VVMC_LKATOIAct_enum"
  VVMC_LKATOIAct_enum_Inproc/1 -> UnitConverter579/1
  UnitConverter579/1 -> VOUTP_LKATOIAct_enum/1  "VOUTP_LKATOIAct_enum"
  VVMC_ADASAEBReq_enum/1 -> VVMC_ADASAEBReq_enum_Inproc/1  "VVMC_ADASAEBReq_enum"
  VVMC_ADASAEBReq_enum_Inproc/1 -> UnitConverter580/1
  UnitConverter580/1 -> VOUTP_ADASAEBReq_enum/1  "VOUTP_ADASAEBReq_enum"
  VVMC_ADASFaultSta_flg/1 -> VVMC_ADASFaultSta_flg_Inproc/1  "VVMC_ADASFaultSta_flg"
  VVMC_ADASFaultSta_flg_Inproc/1 -> UnitConverter581/1
  UnitConverter581/1 -> VOUTP_ADASFaultSta_flg/1  "VOUTP_ADASFaultSta_flg"
  VVMC_AEBVehHoldReq_flg/1 -> VVMC_AEBVehHoldReq_flg_Inproc/1  "VVMC_AEBVehHoldReq_flg"
  VVMC_AEBVehHoldReq_flg_Inproc/1 -> UnitConverter582/1
  UnitConverter582/1 -> VOUTP_AEBVehHoldReq_flg/1  "VOUTP_AEBVehHoldReq_flg"
  VVMC_ACCVehHoldReq_flg/1 -> VVMC_ACCVehHoldReq_flg_Inproc/1  "VVMC_ACCVehHoldReq_flg"
  VVMC_ACCVehHoldReq_flg_Inproc/1 -> UnitConverter583/1
  UnitConverter583/1 -> VOUTP_ACCVehHoldReq_flg/1  "VOUTP_ACCVehHoldReq_flg"
  VVMC_ADASDBSReq_enum/1 -> VVMC_ADASDBSReq_enum_Inproc/1  "VVMC_ADASDBSReq_enum"
  VVMC_ADASDBSReq_enum_Inproc/1 -> UnitConverter584/1
  UnitConverter584/1 -> VOUTP_ADASDBSReq_enum/1  "VOUTP_ADASDBSReq_enum"
  VVMC_ADASACCSta_enum/1 -> VVMC_ADASACCSta_enum_Inproc/1  "VVMC_ADASACCSta_enum"
  VVMC_ADASACCSta_enum_Inproc/1 -> UnitConverter585/1
  UnitConverter585/1 -> VOUTP_ADASACCSta_enum/1  "VOUTP_ADASACCSta_enum"
  VVMC_ACCObjDist_m/1 -> VVMC_ACCObjDist_m_Inproc/1  "VVMC_ACCObjDist_m"
  VVMC_ACCObjDist_m_Inproc/1 -> UnitConverter586/1
  UnitConverter586/1 -> VOUTP_ACCObjDist_m/1  "VOUTP_ACCObjDist_m"
  VVMC_ACCObjRelSpd_mps/1 -> VVMC_ACCObjRelSpd_mps_Inproc/1  "VVMC_ACCObjRelSpd_mps"
  VVMC_ACCObjRelSpd_mps_Inproc/1 -> UnitConverter587/1
  UnitConverter587/1 -> VOUTP_ACCObjRelSpd_mps/1  "VOUTP_ACCObjRelSpd_mps"
  VVMC_TimeGapLevel_enum/1 -> VVMC_TimeGapLevel_enum_Inproc/1  "VVMC_TimeGapLevel_enum"
  VVMC_TimeGapLevel_enum_Inproc/1 -> UnitConverter588/1
  UnitConverter588/1 -> VOUTP_TimeGapLevel_enum/1  "VOUTP_TimeGapLevel_enum"
  VVMC_ACCJerkUpperLimit_mps3/1 -> VVMC_ACCJerkUpperLimit_mps3_Inproc/1  "VVMC_ACCJerkUpperLimit_mps3"
  VVMC_ACCJerkUpperLimit_mps3_Inproc/1 -> UnitConverter589/1
  UnitConverter589/1 -> VOUTP_ACCJerkUpperLimit_mps3/1  "VOUTP_ACCJerkUpperLimit_mps3"
  VVMC_ACCComfortBandUpper_mps2/1 -> VVMC_ACCComfortBandUpper_mps2_Inproc/1  "VVMC_ACCComfortBandUpper_mps2"
  VVMC_ACCComfortBandUpper_mps2_Inproc/1 -> UnitConverter590/1
  UnitConverter590/1 -> VOUTP_ACCComfortBandUpper_mps2/1  "VOUTP_ACCComfortBandUpper_mps2"
  VVMC_ACCJerkLowerLimit_mps3/1 -> VVMC_ACCJerkLowerLimit_mps3_Inproc/1  "VVMC_ACCJerkLowerLimit_mps3"
  VVMC_ACCJerkLowerLimit_mps3_Inproc/1 -> UnitConverter591/1
  UnitConverter591/1 -> VOUTP_ACCJerkLowerLimit_mps3/1  "VOUTP_ACCJerkLowerLimit_mps3"
  VVMC_ACCComfortBandLower_mps2/1 -> VVMC_ACCComfortBandLower_mps2_Inproc/1  "VVMC_ACCComfortBandLower_mps2"
  VVMC_ACCComfortBandLower_mps2_Inproc/1 -> UnitConverter592/1
  UnitConverter592/1 -> VOUTP_ACCComfortBandLower_mps2/1  "VOUTP_ACCComfortBandLower_mps2"
  VVMC_ADASVehSpdLim_raw32/1 -> VVMC_ADASVehSpdLim_raw32_Inproc/1  "VVMC_ADASVehSpdLim_raw32"
  VVMC_ADASVehSpdLim_raw32_Inproc/1 -> UnitConverter593/1
  UnitConverter593/1 -> VOUTP_ADASVehSpdLim_raw32/1  "VOUTP_ADASVehSpdLim_raw32"
  VVMC_ADASShftPosnReqA_flg/1 -> VVMC_ADASShftPosnReqA_flg_Inproc/1  "VVMC_ADASShftPosnReqA_flg"
  VVMC_ADASShftPosnReqA_flg_Inproc/1 -> UnitConverter594/1
  UnitConverter594/1 -> VOUTP_ADASShftPosnReqA_flg/1  "VOUTP_ADASShftPosnReqA_flg"
  VVMC_ADASShftPosnReq_enum/1 -> VVMC_ADASShftPosnReq_enum_Inproc/1  "VVMC_ADASShftPosnReq_enum"
  VVMC_ADASShftPosnReq_enum_Inproc/1 -> UnitConverter595/1
  UnitConverter595/1 -> VOUTP_ADASShftPosnReq_enum/1  "VOUTP_ADASShftPosnReq_enum"
  VVMC_ADASForceIdle_flg/1 -> VVMC_ADASForceIdle_flg_Inproc/1  "VVMC_ADASForceIdle_flg"
  VVMC_ADASForceIdle_flg_Inproc/1 -> UnitConverter596/1
  UnitConverter596/1 -> VOUTP_ADASForceIdle_flg/1  "VOUTP_ADASForceIdle_flg"
  VVMC_HazardWarningReq_flg/1 -> VVMC_HazardWarningReq_flg_Inproc/1  "VVMC_HazardWarningReq_flg"
  VVMC_HazardWarningReq_flg_Inproc/1 -> UnitConverter597/1
  UnitConverter597/1 -> VOUTP_HazardWarningReq_flg/1  "VOUTP_HazardWarningReq_flg"
  VVMC_RightTurnLightReq_flg/1 -> VVMC_RightTurnLightReq_flg_Inproc/1  "VVMC_RightTurnLightReq_flg"
  VVMC_RightTurnLightReq_flg_Inproc/1 -> UnitConverter598/1
  UnitConverter598/1 -> VOUTP_RightTurnLightReq_flg/1  "VOUTP_RightTurnLightReq_flg"
  VVMC_LeftTurnLightReq_flg/1 -> VVMC_LeftTurnLightReq_flg_Inproc/1  "VVMC_LeftTurnLightReq_flg"
  VVMC_LeftTurnLightReq_flg_Inproc/1 -> UnitConverter599/1
  UnitConverter599/1 -> VOUTP_LeftTurnLightReq_flg/1  "VOUTP_LeftTurnLightReq_flg"
  VVMC_ADASFCWSta_enum/1 -> VVMC_ADASFCWSta_enum_Inproc/1  "VVMC_ADASFCWSta_enum"
  VVMC_ADASFCWSta_enum_Inproc/1 -> UnitConverter600/1
  UnitConverter600/1 -> VOUTP_ADASFCWSta_enum/1  "VOUTP_ADASFCWSta_enum"
  VVMC_ADASLDWSta_enum/1 -> VVMC_ADASLDWSta_enum_Inproc/1  "VVMC_ADASLDWSta_enum"
  VVMC_ADASLDWSta_enum_Inproc/1 -> UnitConverter601/1
  UnitConverter601/1 -> VOUTP_ADASLDWSta_enum/1  "VOUTP_ADASLDWSta_enum"
  VVMC_ADASFltWrnReq_flg/1 -> VVMC_ADASFltWrnReq_flg_Inproc/1  "VVMC_ADASFltWrnReq_flg"
  VVMC_ADASFltWrnReq_flg_Inproc/1 -> UnitConverter602/1
  UnitConverter602/1 -> VOUTP_ADASFltWrnReq_flg/1  "VOUTP_ADASFltWrnReq_flg"
  VVMC_ACCObjDstLvl_enum/1 -> VVMC_ACCObjDstLvl_enum_Inproc/1  "VVMC_ACCObjDstLvl_enum"
  VVMC_ACCObjDstLvl_enum_Inproc/1 -> UnitConverter603/1
  UnitConverter603/1 -> VOUTP_ACCObjDstLvl_enum/1  "VOUTP_ACCObjDstLvl_enum"
  VVMC_ForceLowBeam_enum/1 -> VVMC_ForceLowBeam_enum_Inproc/1  "VVMC_ForceLowBeam_enum"
  VVMC_ForceLowBeam_enum_Inproc/1 -> UnitConverter604/1
  UnitConverter604/1 -> VOUTP_ForceLowBeam_enum/1  "VOUTP_ForceLowBeam_enum"
  VVMC_ACCTakeoverReq_flg/1 -> VVMC_ACCTakeoverReq_flg_Inproc/1  "VVMC_ACCTakeoverReq_flg"
  VVMC_ACCTakeoverReq_flg_Inproc/1 -> UnitConverter605/1
  UnitConverter605/1 -> VOUTP_ACCTakeoverReq_flg/1  "VOUTP_ACCTakeoverReq_flg"
  VVMC_ADASWarningMsg_enum/1 -> VVMC_ADASWarningMsg_enum_Inproc/1  "VVMC_ADASWarningMsg_enum"
  VVMC_ADASWarningMsg_enum_Inproc/1 -> UnitConverter606/1
  UnitConverter606/1 -> VOUTP_ADASWarningMsg_enum/1  "VOUTP_ADASWarningMsg_enum"
  VVMC_ADASCAMSpdLim_enum/1 -> VVMC_ADASCAMSpdLim_enum_Inproc/1  "VVMC_ADASCAMSpdLim_enum"
  VVMC_ADASCAMSpdLim_enum_Inproc/1 -> UnitConverter607/1
  UnitConverter607/1 -> VOUTP_ADASCAMSpdLim_enum/1  "VOUTP_ADASCAMSpdLim_enum"
  VVMC_TargetType_enum/1 -> VVMC_TargetType_enum_Inproc/1  "VVMC_TargetType_enum"
  VVMC_TargetType_enum_Inproc/1 -> UnitConverter608/1
  UnitConverter608/1 -> VOUTP_TargetType_enum/1  "VOUTP_TargetType_enum"
  VVMC_ADASSLIFSpdLim_enum/1 -> VVMC_ADASSLIFSpdLim_enum_Inproc/1  "VVMC_ADASSLIFSpdLim_enum"
  VVMC_ADASSLIFSpdLim_enum_Inproc/1 -> UnitConverter609/1
  UnitConverter609/1 -> VOUTP_ADASSLIFSpdLim_enum/1  "VOUTP_ADASSLIFSpdLim_enum"
  VVMC_LKAHODDisplayWarning_flg/1 -> VVMC_LKAHODDisplayWarning_flg_Inproc/1  "VVMC_LKAHODDisplayWarning_flg"
  VVMC_LKAHODDisplayWarning_flg_Inproc/1 -> UnitConverter610/1
  UnitConverter610/1 -> VOUTP_LKAHODDisplayWarning_flg/1  "VOUTP_LKAHODDisplayWarning_flg"
  VVMC_LKAHODSoundWarning_flg/1 -> VVMC_LKAHODSoundWarning_flg_Inproc/1  "VVMC_LKAHODSoundWarning_flg"
  VVMC_LKAHODSoundWarning_flg_Inproc/1 -> UnitConverter611/1
  UnitConverter611/1 -> VOUTP_LKAHODSoundWarning_flg/1  "VOUTP_LKAHODSoundWarning_flg"
  VVMC_ADASLFCSta_enum/1 -> VVMC_ADASLFCSta_enum_Inproc/1  "VVMC_ADASLFCSta_enum"
  VVMC_ADASLFCSta_enum_Inproc/1 -> UnitConverter612/1
  UnitConverter612/1 -> VOUTP_ADASLFCSta_enum/1  "VOUTP_ADASLFCSta_enum"
  VVMC_ADASLaneModeL_enum/1 -> VVMC_ADASLaneModeL_enum_Inproc/1  "VVMC_ADASLaneModeL_enum"
  VVMC_ADASLaneModeL_enum_Inproc/1 -> UnitConverter613/1
  UnitConverter613/1 -> VOUTP_ADASLaneModeL_enum/1  "VOUTP_ADASLaneModeL_enum"
  VVMC_ADASLaneModeR_enum/1 -> VVMC_ADASLaneModeR_enum_Inproc/1  "VVMC_ADASLaneModeR_enum"
  VVMC_ADASLaneModeR_enum_Inproc/1 -> UnitConverter614/1
  UnitConverter614/1 -> VOUTP_ADASLaneModeR_enum/1  "VOUTP_ADASLaneModeR_enum"
  VVMC_ADASSLIFSta_enum/1 -> VVMC_ADASSLIFSta_enum_Inproc/1  "VVMC_ADASSLIFSta_enum"
  VVMC_ADASSLIFSta_enum_Inproc/1 -> UnitConverter615/1
  UnitConverter615/1 -> VOUTP_ADASSLIFSta_enum/1  "VOUTP_ADASSLIFSta_enum"
  VVMC_ADASISASta_enum/1 -> VVMC_ADASISASta_enum_Inproc/1  "VVMC_ADASISASta_enum"
  VVMC_ADASISASta_enum_Inproc/1 -> UnitConverter616/1
  UnitConverter616/1 -> VOUTP_ADASISASta_enum/1  "VOUTP_ADASISASta_enum"
  VVMC_ADASLDWMute_flg/1 -> VVMC_ADASLDWMute_flg_Inproc/1  "VVMC_ADASLDWMute_flg"
  VVMC_ADASLDWMute_flg_Inproc/1 -> UnitConverter617/1
  UnitConverter617/1 -> VOUTP_ADASLDWMute_flg/1  "VOUTP_ADASLDWMute_flg"
  VVMC_ADASFCWMute_flg/1 -> VVMC_ADASFCWMute_flg_Inproc/1  "VVMC_ADASFCWMute_flg"
  VVMC_ADASFCWMute_flg_Inproc/1 -> UnitConverter618/1
  UnitConverter618/1 -> VOUTP_ADASFCWMute_flg/1  "VOUTP_ADASFCWMute_flg"
  VVMC_ADASLFCHandsOffWarning_enum/1 -> VVMC_ADASLFCHandsOffWarning_enum_Inproc/1  "VVMC_ADASLFCHandsOffWarning_enum"
  VVMC_ADASLFCHandsOffWarning_enum_Inproc/1 -> UnitConverter619/1
  UnitConverter619/1 -> VOUTP_ADASLFCHandsOffWarning_enum/1  "VOUTP_ADASLFCHandsOffWarning_enum"
  VVMC_LVDADisabled_flg/1 -> VVMC_LVDADisabled_flg_Inproc/1  "VVMC_LVDADisabled_flg"
  VVMC_LVDADisabled_flg_Inproc/1 -> UnitConverter620/1
  UnitConverter620/1 -> VOUTP_LVDADisabled_flg/1  "VOUTP_LVDADisabled_flg"
  VVMC_LVDAMuteSta_enum/1 -> VVMC_LVDAMuteSta_enum_Inproc/1  "VVMC_LVDAMuteSta_enum"
  VVMC_LVDAMuteSta_enum_Inproc/1 -> UnitConverter621/1
  UnitConverter621/1 -> VOUTP_LVDAMuteSta_enum/1  "VOUTP_LVDAMuteSta_enum"
  VVMC_LVDAFailinfo_flg/1 -> VVMC_LVDAFailinfo_flg_Inproc/1  "VVMC_LVDAFailinfo_flg"
  VVMC_LVDAFailinfo_flg_Inproc/1 -> UnitConverter622/1
  UnitConverter622/1 -> VOUTP_LVDAFailinfo_flg/1  "VOUTP_LVDAFailinfo_flg"
  VVMC_LVDAWarning_flg/1 -> VVMC_LVDAWarning_flg_Inproc/1  "VVMC_LVDAWarning_flg"
  VVMC_LVDAWarning_flg_Inproc/1 -> UnitConverter623/1
  UnitConverter623/1 -> VOUTP_LVDAWarning_flg/1  "VOUTP_LVDAWarning_flg"
  VVMC_LVDAACCStatusInformation_flg/1 -> VVMC_LVDAACCStatusInformation_flg_Inproc/1  "VVMC_LVDAACCStatusInformation_flg"
  VVMC_LVDAACCStatusInformation_flg_Inproc/1 -> UnitConverter624/1
  UnitConverter624/1 -> VOUTP_LVDAACCStatusInformation_flg/1  "VOUTP_LVDAACCStatusInformation_flg"
  VVMC_ADASLFCWarnSound_enum/1 -> VVMC_ADASLFCWarnSound_enum_Inproc/1  "VVMC_ADASLFCWarnSound_enum"
  VVMC_ADASLFCWarnSound_enum_Inproc/1 -> UnitConverter625/1
  UnitConverter625/1 -> VOUTP_ADASLFCWarnSound_enum/1  "VOUTP_ADASLFCWarnSound_enum"
  VVMC_FCMACCmode_enum/1 -> VVMC_FCMACCmode_enum_Inproc/1  "VVMC_FCMACCmode_enum"
  VVMC_FCMACCmode_enum_Inproc/1 -> UnitConverter626/1
  UnitConverter626/1 -> VOUTP_FCMACCmode_enum/1  "VOUTP_FCMACCmode_enum"
  VVMC_ADASLanetypeR_enum/1 -> VVMC_ADASLanetypeR_enum_Inproc/1  "VVMC_ADASLanetypeR_enum"
  VVMC_ADASLanetypeR_enum_Inproc/1 -> UnitConverter627/1
  UnitConverter627/1 -> VOUTP_ADASLanetypeR_enum/1  "VOUTP_ADASLanetypeR_enum"
  VVMC_ADASLanetypeL_enum/1 -> VVMC_ADASLanetypeL_enum_Inproc/1  "VVMC_ADASLanetypeL_enum"
  VVMC_ADASLanetypeL_enum_Inproc/1 -> UnitConverter628/1
  UnitConverter628/1 -> VOUTP_ADASLanetypeL_enum/1  "VOUTP_ADASLanetypeL_enum"
  VVMC_ADASLanecurveL_raw32/1 -> VVMC_ADASLanecurveL_raw32_Inproc/1  "VVMC_ADASLanecurveL_raw32"
  VVMC_ADASLanecurveL_raw32_Inproc/1 -> UnitConverter629/1
  UnitConverter629/1 -> VOUTP_ADASLanecurveL_raw32/1  "VOUTP_ADASLanecurveL_raw32"
  VVMC_ADASLanecurveR_raw32/1 -> VVMC_ADASLanecurveR_raw32_Inproc/1  "VVMC_ADASLanecurveR_raw32"
  VVMC_ADASLanecurveR_raw32_Inproc/1 -> UnitConverter630/1
  UnitConverter630/1 -> VOUTP_ADASLanecurveR_raw32/1  "VOUTP_ADASLanecurveR_raw32"
  VVMC_ADASAEBSta_enum/1 -> VVMC_ADASAEBSta_enum_Inproc/1  "VVMC_ADASAEBSta_enum"
  VVMC_ADASAEBSta_enum_Inproc/1 -> UnitConverter631/1
  UnitConverter631/1 -> VOUTP_ADASAEBSta_enum/1  "VOUTP_ADASAEBSta_enum"
  VVMC_FCMLDWRequest_enum/1 -> VVMC_FCMLDWRequest_enum_Inproc/1  "VVMC_FCMLDWRequest_enum"
  VVMC_FCMLDWRequest_enum_Inproc/1 -> UnitConverter632/1
  UnitConverter632/1 -> VOUTP_FCMLDWRequest_enum/1  "VOUTP_FCMLDWRequest_enum"
  VVMC_FCMLDWFault_flg/1 -> VVMC_FCMLDWFault_flg_Inproc/1  "VVMC_FCMLDWFault_flg"
  VVMC_FCMLDWFault_flg_Inproc/1 -> UnitConverter633/1
  UnitConverter633/1 -> VOUTP_FCMLDWFault_flg/1  "VOUTP_FCMLDWFault_flg"
  VVMC_ACCCtrlAvail_flg/1 -> VVMC_ACCCtrlAvail_flg_Inproc/1  "VVMC_ACCCtrlAvail_flg"
  VVMC_ACCCtrlAvail_flg_Inproc/1 -> UnitConverter634/1
  UnitConverter634/1 -> VOUTP_ACCCtrlAvail_flg/1  "VOUTP_ACCCtrlAvail_flg"
  VVMC_ACCPedalOvrd_flg/1 -> VVMC_ACCPedalOvrd_flg_Inproc/1  "VVMC_ACCPedalOvrd_flg"
  VVMC_ACCPedalOvrd_flg_Inproc/1 -> UnitConverter635/1
  UnitConverter635/1 -> VOUTP_ACCPedalOvrd_flg/1  "VOUTP_ACCPedalOvrd_flg"
  VVMC_TimeGapCalcu_s/1 -> VVMC_TimeGapCalcu_s_Inproc/1  "VVMC_TimeGapCalcu_s"
  VVMC_TimeGapCalcu_s_Inproc/1 -> UnitConverter636/1
  UnitConverter636/1 -> VOUTP_TimeGapCalcu_s/1  "VOUTP_TimeGapCalcu_s"
  VVMC_CCCtrlSta_enum/1 -> VVMC_CCCtrlSta_enum_Inproc/1  "VVMC_CCCtrlSta_enum"
  VVMC_CCCtrlSta_enum_Inproc/1 -> UnitConverter637/1
  UnitConverter637/1 -> VOUTP_CCCtrlSta_enum/1  "VOUTP_CCCtrlSta_enum"
  VVMC_MSACtrlSta_enum/1 -> VVMC_MSACtrlSta_enum_Inproc/1  "VVMC_MSACtrlSta_enum"
  VVMC_MSACtrlSta_enum_Inproc/1 -> UnitConverter638/1
  UnitConverter638/1 -> VOUTP_MSACtrlSta_enum/1  "VOUTP_MSACtrlSta_enum"
  VVMC_APSCtrlAvail_flg/1 -> VVMC_APSCtrlAvail_flg_Inproc/1  "VVMC_APSCtrlAvail_flg"
  VVMC_APSCtrlAvail_flg_Inproc/1 -> UnitConverter639/1
  UnitConverter639/1 -> VOUTP_APSCtrlAvail_flg/1  "VOUTP_APSCtrlAvail_flg"
  VVMC_APSStaSys_enum/1 -> VVMC_APSStaSys_enum_Inproc/1  "VVMC_APSStaSys_enum"
  VVMC_APSStaSys_enum_Inproc/1 -> UnitConverter640/1
  UnitConverter640/1 -> VOUTP_APSStaSys_enum/1  "VOUTP_APSStaSys_enum"
  VVMC_APSDecReqA_flg/1 -> VVMC_APSDecReqA_flg_Inproc/1  "VVMC_APSDecReqA_flg"
  VVMC_APSDecReqA_flg_Inproc/1 -> UnitConverter641/1
  UnitConverter641/1 -> VOUTP_APSDecReqA_flg/1  "VOUTP_APSDecReqA_flg"
  VVMC_APSDecReq_mps2/1 -> VVMC_APSDecReq_mps2_Inproc/1  "VVMC_APSDecReq_mps2"
  VVMC_APSDecReq_mps2_Inproc/1 -> UnitConverter642/1
  UnitConverter642/1 -> VOUTP_APSDecReq_mps2/1  "VOUTP_APSDecReq_mps2"
  VVMC_APSReq_enum/1 -> VVMC_APSReq_enum_Inproc/1  "VVMC_APSReq_enum"
  VVMC_APSReq_enum_Inproc/1 -> UnitConverter643/1
  UnitConverter643/1 -> VOUTP_APSReq_enum/1  "VOUTP_APSReq_enum"
  VVMC_CCMSASpdWar_flg/1 -> VVMC_CCMSASpdWar_flg_Inproc/1  "VVMC_CCMSASpdWar_flg"
  VVMC_CCMSASpdWar_flg_Inproc/1 -> UnitConverter644/1
  UnitConverter644/1 -> VOUTP_CCMSASpdWar_flg/1  "VOUTP_CCMSASpdWar_flg"
  VVMC_IMUEnaCmd_flg/1 -> VVMC_IMUEnaCmd_flg_Inproc/1  "VVMC_IMUEnaCmd_flg"
  VVMC_IMUEnaCmd_flg_Inproc/1 -> UnitConverter645/1
  UnitConverter645/1 -> VOUTP_IMUEnaCmd_flg/1  "VOUTP_IMUEnaCmd_flg"
